simulink model "Project_UR5"  (Simulink 8.3)
settings: Solver=ode3  StartTime=0.0  StopTime=tf  FixedStep=ts  RelTol=1e-3
values from neighbouring files (symbols this model uses):
  qi = [0;pi/4;0;-pi/3;0;0]    [initial.m]
(part 2 of 3)

== matlab function Inverse Kinematics & Redundant Kinematic Controller ==
  data: x_des input double; dq output double; xd_des input double; q input double
function dq = IK_Control(x_des,xd_des,q)
%Input Decomposition
q1 = q(1);
q2 = q(2);
q3 = q(3);
q4 = q(4);
q5 = q(5);
q6 = q(6);
%% %% Inverse Kinematics
%% End Effector Position
x = [(379*cos(q2 + q3)*cos(q1)*sin(q4))/4 - 425*cos(q1)*cos(q2) - (165*cos(q5)*sin(q1))/2 - (165*cos(q2 + q3 + q4)*cos(q1)*sin(q5))/2 - (1093*sin(q1))/10 + (379*sin(q2 + q3)*cos(q1)*cos(q4))/4 - 392*cos(q1)*cos(q2)*cos(q3) + 392*cos(q1)*sin(q2)*sin(q3);
(1093*cos(q1))/10 + (165*cos(q1)*cos(q5))/2 - 425*cos(q2)*sin(q1) + 392*sin(q1)*sin(q2)*sin(q3) - (165*cos(q2 + q3 + q4)*sin(q1)*sin(q5))/2 + (379*cos(q2 + q3)*sin(q1)*sin(q4))/4 + (379*sin(q2 + q3)*cos(q4)*sin(q1))/4 - 392*cos(q2)*cos(q3)*sin(q1);
392*sin(q2 + q3) + 425*sin(q2) + sin(q5)*((165*cos(q2 + q3)*sin(q4))/2 + (165*sin(q2 + q3)*cos(q4))/2) + (379*cos(q2 + q3)*cos(q4))/4 - (379*sin(q2 + q3)*sin(q4))/4 + 446/5];

%% Jacobian 6x6
J = [ 425*cos(q2)*sin(q1) - (165*cos(q1)*cos(q5))/2 - (1093*cos(q1))/10 - 392*sin(q1)*sin(q2)*sin(q3) + (165*cos(q2 + q3 + q4)*sin(q1)*sin(q5))/2 - (379*cos(q2 + q3)*sin(q1)*sin(q4))/4 - (379*sin(q2 + q3)*cos(q4)*sin(q1))/4 + 392*cos(q2)*cos(q3)*sin(q1), cos(q1)*(392*sin(q2 + q3) + 425*sin(q2) + sin(q5)*((165*cos(q2 + q3)*sin(q4))/2 + (165*sin(q2 + q3)*cos(q4))/2) + (379*cos(q2 + q3)*cos(q4))/4 - (379*sin(q2 + q3)*sin(q4))/4),                     cos(q1)*((379*cos(q2 + q3 + q4))/4 + 392*sin(q2 + q3) + (165*sin(q2 + q3 + q4)*sin(q5))/2),                     cos(q1)*((379*cos(q2 + q3 + q4))/4 + (165*sin(q2 + q3 + q4)*sin(q5))/2), (165*sin(q1)*sin(q5))/2 - (165*cos(q1)*cos(q2)*cos(q3)*cos(q4)*cos(q5))/2 + (165*cos(q1)*cos(q2)*cos(q5)*sin(q3)*sin(q4))/2 + (165*cos(q1)*cos(q3)*cos(q5)*sin(q2)*sin(q4))/2 + (165*cos(q1)*cos(q4)*cos(q5)*sin(q2)*sin(q3))/2,                                                     0;
 (379*cos(q2 + q3)*cos(q1)*sin(q4))/4 - 425*cos(q1)*cos(q2) - (165*cos(q5)*sin(q1))/2 - (165*cos(q2 + q3 + q4)*cos(q1)*sin(q5))/2 - (1093*sin(q1))/10 + (379*sin(q2 + q3)*cos(q1)*cos(q4))/4 - 392*cos(q1)*cos(q2)*cos(q3) + 392*cos(q1)*sin(q2)*sin(q3), sin(q1)*(392*sin(q2 + q3) + 425*sin(q2) + sin(q5)*((165*cos(q2 + q3)*sin(q4))/2 + (165*sin(q2 + q3)*cos(q4))/2) + (379*cos(q2 + q3)*cos(q4))/4 - (379*sin(q2 + q3)*sin(q4))/4),                     sin(q1)*((379*cos(q2 + q3 + q4))/4 + 392*sin(q2 + q3) + (165*sin(q2 + q3 + q4)*sin(q5))/2),                     sin(q1)*((379*cos(q2 + q3 + q4))/4 + (165*sin(q2 + q3 + q4)*sin(q5))/2), (165*cos(q2)*cos(q5)*sin(q1)*sin(q3)*sin(q4))/2 - (165*cos(q2)*cos(q3)*cos(q4)*cos(q5)*sin(q1))/2 - (165*cos(q1)*sin(q5))/2 + (165*cos(q3)*cos(q5)*sin(q1)*sin(q2)*sin(q4))/2 + (165*cos(q4)*cos(q5)*sin(q1)*sin(q2)*sin(q3))/2,                                                     0;
                                                                                                                                                                                                                                                       0,                                                   (165*sin(q2 + q3 + q4 + q5))/4 - (379*sin(q2 + q3 + q4))/4 + 392*cos(q2 + q3) + 425*cos(q2) - (165*sin(q2 + q3 + q4 - q5))/4, (165*sin(q2 + q3 + q4 + q5))/4 - (379*sin(q2 + q3 + q4))/4 + 392*cos(q2 + q3) - (165*sin(q2 + q3 + q4 - q5))/4, (165*sin(q2 + q3 + q4 + q5))/4 - (379*sin(q2 + q3 + q4))/4 - (165*sin(q2 + q3 + q4 - q5))/4,                                                                                                                                                                 (165*sin(q2 + q3 + q4 + q5))/4 + (165*sin(q2 + q3 + q4 - q5))/4,                                                     0;
                                                                                                                                                                                                                                                       0,                                                                                                                                                                       -sin(q1),                                                                                                       -sin(q1),                                                                                    -sin(q1),                                                                                                                                                                                                       sin(q2 + q3 + q4)*cos(q1), - cos(q5)*sin(q1) - cos(q2 + q3 + q4)*cos(q1)*sin(q5);
                                                                                                                                                                                                                                                       0,                                                                                                                                                                        cos(q1),                                                                                                        cos(q1),                                                                                     cos(q1),                                                                                                                                                                                                       sin(q2 + q3 + q4)*sin(q1),   cos(q1)*cos(q5) - cos(q2 + q3 + q4)*sin(q1)*sin(q5);
                                                                                                                                                                                                                                                       1,                                                                                                                                                                              0,                                                                                                              0,                                                                                           0,                                                                                                                                                                                                               cos(q2 + q3 + q4),                             sin(q2 + q3 + q4)*sin(q5)];

%% Redundant Jacobian 3x6
Jp=J(1:3,1:6) ; %% Task only takes 3 DOFs to control x,y,z.

% %% manipulability measure #1: W=det(Jp*Jp.')
% kp=0.001;
% dq0=[0;
%    -(2^(1/2)*(317026377437840000*cos(2*q2 + q4) - 1082343818118750000*cos(2*q2 - q3 - q4 - q5) - 41912575773750000*cos(2*q2 - q3 - q4 - 2*q5) + 16565733236250000*cos(2*q2 - q3 - q4 + 2*q5) - 540213828000000000*cos(2*q2 - 2*q3 - q4 - q5) + 396576415666421760*cos(2*q2 + 2*q3 - q4 - q5) + 16552357593750000*cos(2*q2 - q3 - q4 - 3*q5) - 16552357593750000*cos(2*q2 - q3 - q4 + 3*q5) - 45886635629936640*cos(2*q2 + 2*q3 - q4 - 2*q5) + 45886635629936640*cos(2*q2 + 2*q3 - q4 + 2*q5) + 17317691854848000*cos(2*q2 + 2*q3 - q4 - 3*q5) - 17317691854848000*cos(2*q2 + 2*q3 - q4 + 3*q5) + 192863414377307520*cos(2*q2 + 2*q3 + 3*q4 - q5) + 139667883829911360*cos(2*q2 + 2*q3 + 3*q4 - 2*q5) + 136338643638267840*cos(2*q2 + 2*q3 + 3*q4 + 2*q5) + 275626326313503000*cos(2*q2 + 3*q3 + 3*q4 - q5) + 34919056932883200*cos(2*q2 + 2*q3 + 3*q4 - 3*q5) - 30250558196812800*cos(2*q2 + 2*q3 + 3*q4 + 3*q5) + 175870104928699500*cos(2*q2 + 3*q3 + 3*q4 - 2*q5) + 174065350998280500*cos(2*q2 + 3*q3 + 3*q4 + 2*q5) + 200938795318800000*cos(2*q2 + 4*q3 + 3*q4 - q5) + 508114967976000*cos(2*q2 + 2*q3 + 3*q4 - 4*q5) - 508114967976000*cos(2*q2 + 2*q3 + 3*q4 + 4*q5) + 36593293892265000*cos(2*q2 + 3*q3 + 3*q4 - 3*q5) - 34062538837635000*cos(2*q2 + 3*q3 + 3*q4 + 3*q5) + 116893673820000000*cos(2*q2 + 4*q3 + 3*q4 - 2*q5) + 116893673820000000*cos(2*q2 + 4*q3 + 3*q4 + 2*q5) + 275444976262500*cos(2*q2 + 3*q3 + 3*q4 - 4*q5) - 275444976262500*cos(2*q2 + 3*q3 + 3*q4 + 4*q5) + 20356154280000000*cos(2*q2 + 4*q3 + 3*q4 - 3*q5) - 20356154280000000*cos(2*q2 + 4*q3 + 3*q4 + 3*q5) + 14526380593972122400*sin(2*q2 + q3) - 4445768516062500*sin(2*q2 + q5) - 722615438160000000*sin(2*q2 - q3 - 2*q4 - q5) + 262162593000000000*sin(2*q2 - q3 - 2*q4 - 2*q5) + 262162593000000000*sin(2*q2 - q3 - 2*q4 + 2*q5) - 261149286750000000*sin(2*q2 - 2*q3 - 2*q4 - q5) - 189006783727534080*sin(2*q2 + 2*q3 - 2*q4 - q5) + 127716498108106380*sin(2*q2 + 2*q3 + 2*q4 - q5) + 85269720937500000*sin(2*q2 - 2*q3 - 2*q4 - 2*q5) + 85269720937500000*sin(2*q2 - 2*q3 - 2*q4 + 2*q5) + 82285275237580800*sin(2*q2 + 2*q3 - 2*q4 - 2*q5) + 82285275237580800*sin(2*q2 + 2*q3 - 2*q4 + 2*q5) + 235845517878338346*sin(2*q2 + 2*q3 + 2*q4 - 2*q5) + 165406186902402666*sin(2*q2 + 2*q3 + 2*q4 + 2*q5) + 1142121750227304000*sin(2*q2 + 3*q3 + 2*q4 - q5) + 18769510446883020*sin(2*q2 + 2*q3 + 2*q4 - 3*q5) + 11896689054513780*sin(2*q2 + 2*q3 + 2*q4 + 3*q5) - 11620198292989440*sin(2*q2 + 2*q3 + 4*q4 - q5) + 358818080264028000*sin(2*q2 + 3*q3 + 2*q4 - 2*q5) + 334768238290332000*sin(2*q2 + 3*q3 + 2*q4 + 2*q5) + 777590887180800000*sin(2*q2 + 4*q3 + 2*q4 - q5) + 748031352071850*sin(2*q2 + 2*q3 + 2*q4 - 4*q5) + 748031352071850*sin(2*q2 + 2*q3 + 2*q4 + 4*q5) - 15003495465235200*sin(2*q2 + 2*q3 + 4*q4 - 2*q5) - 15003495465235200*sin(2*q2 + 2*q3 + 4*q4 + 2*q5) + 5235123912480000*sin(2*q2 + 3*q3 + 2*q4 - 3*q5) + 5235123912480000*sin(2*q2 + 3*q3 + 2*q4 + 3*q5) - 12598429271736000*sin(2*q2 + 3*q3 + 4*q4 - q5) + 193445150976000000*sin(2*q2 + 4*q3 + 2*q4 - 2*q5) + 193445150976000000*sin(2*q2 + 4*q3 + 2*q4 + 2*q5) - 6278767742016000*sin(2*q2 + 2*q3 + 4*q4 - 3*q5) + 6278767742016000*sin(2*q2 + 2*q3 + 4*q4 + 3*q5) - 16266544828380000*sin(2*q2 + 3*q3 + 4*q4 - 2*q5) - 16266544828380000*sin(2*q2 + 3*q3 + 4*q4 + 2*q5) - 12428943969337500*sin(2*q2 + 4*q3 + 4*q4 - q5) - 911166822720000*sin(2*q2 + 2*q3 + 4*q4 - 4*q5) - 911166822720000*sin(2*q2 + 2*q3 + 4*q4 + 4*q5) - 6807337475400000*sin(2*q2 + 3*q3 + 4*q4 - 3*q5) + 6807337475400000*sin(2*q2 + 3*q3 + 4*q4 + 3*q5) - 16223208602906250*sin(2*q2 + 4*q3 + 4*q4 - 2*q5) - 16223208602906250*sin(2*q2 + 4*q3 + 4*q4 + 2*q5) - 987872193000000*sin(2*q2 + 3*q3 + 4*q4 - 4*q5) - 987872193000000*sin(2*q2 + 3*q3 + 4*q4 + 4*q5) - 6150336792187500*sin(2*q2 + 4*q3 + 4*q4 - 3*q5) + 6150336792187500*sin(2*q2 + 4*q3 + 4*q4 + 3*q5) - 803276177343750*sin(2*q2 + 4*q3 + 4*q4 - 4*q5) - 803276177343750*sin(2*q2 + 4*q3 + 4*q4 + 4*q5) + 2498784373190000000*cos(2*q2 - q3 - q4) + 1240854792800000000*cos(2*q2 - 2*q3 - q4) - 871145795906584576*cos(2*q2 + 2*q3 - q4) - 62388715527600000*cos(2*q2 - q4 - q5) + 63675071524036224*cos(2*q2 + 2*q3 + 3*q4) - 92595827847600000*cos(2*q2 - q4 - 2*q5) + 69217093083600000*cos(2*q2 - q4 + 2*q5) + 45801347130000000*cos(2*q2 - q4 - 3*q5) - 45801347130000000*cos(2*q2 - q4 + 3*q5) + 34513957880105600*cos(2*q2 + 3*q3 + 3*q4) - 2008123829040000*cos(2*q2 + 4*q3 + 3*q4) + 4969165728210312500*sin(2*q2) + 725047844808000000*sin(2*q2 - q3 - 2*q4) + 104865037200000000*sin(2*q2 - q3 - 2*q5) + 104865037200000000*sin(2*q2 - q3 + 2*q5) + 243079518400000000*sin(2*q2 - 2*q3 - 2*q4) + 217071427371925504*sin(2*q2 + 2*q3 - 2*q4) + 438536338768182720*sin(2*q2 + 2*q3 + 2*q4) - 11750186456870400*sin(2*q2 + 2*q3 - q5) - 131469808648502016*sin(2*q2 + 2*q3 - 2*q5) - 175834693607037696*sin(2*q2 + 2*q3 + 2*q5) + 1012290445559159200*sin(2*q2 + 3*q3 + 2*q4) - 888675299635200000*sin(2*q2 - 2*q4 - q5) + 333253237363200000*sin(2*q2 + 2*q4 - q5) + 9532529563768064*sin(2*q2 + 2*q3 + 4*q4) + 7564341295526400*sin(2*q2 + 2*q3 - 3*q5) + 11750186456870400*sin(2*q2 + 2*q3 + 3*q5) + 362709658080000000*sin(2*q2 - 2*q4 - 2*q5) + 362709658080000000*sin(2*q2 - 2*q4 + 2*q5) + 120903219360000000*sin(2*q2 + 2*q4 - 2*q5) + 120903219360000000*sin(2*q2 + 2*q4 + 2*q5) + 602883625783040000*sin(2*q2 + 4*q3 + 2*q4) - 1822333645440000*sin(2*q2 + 2*q3 - 4*q5) - 1822333645440000*sin(2*q2 + 2*q3 + 4*q5) + 10335012919901600*sin(2*q2 + 3*q3 + 4*q4) + 13494962268852500*sin(2*q2 + 4*q3 + 4*q4) + 2457973257707649000*cos(2*q2 + q3 + q4 - q5) - 869311129682688000*cos(2*q2 + q3 - q4 + q5) + 498267813120000000*cos(2*q2 - q3 + q4 + q5) - 133864358657663700*cos(2*q2 + q3 + q4 - 2*q5) + 76464939583365300*cos(2*q2 + q3 + q4 + 2*q5) - 1325918940020727360*cos(2*q2 + 2*q3 + q4 + q5) + 689315467203000*cos(2*q2 + q3 + q4 - 3*q5) + 6902949696687000*cos(2*q2 + q3 + q4 + 3*q5) - 129816178829568000*cos(2*q2 + q3 + 3*q4 + q5) + 1407721742617344000*cos(2*q2 + 3*q3 + q4 + q5) + 1377224881312500*cos(2*q2 + q3 + q4 - 4*q5) - 1377224881312500*cos(2*q2 + q3 + q4 + 4*q5) + 919157565849600000*cos(2*q2 + 4*q3 + q4 + q5) + 614754207277056000*sin(2*q2 + q3 - 2*q4 + q5) - 153499453009056000*sin(2*q2 + q3 + 2*q4 + q5) + 225130560673760000*cos(2*q2 - q4) - 5011691754440000000*sin(2*q2 - q3) - 2566834188800000000*sin(2*q2 - 2*q3) + 4963773870401251584*sin(2*q2 + 2*q3) - 4321284125611622400*sin(2*q2 + 3*q3) + 972268829109760000*sin(2*q2 - 2*q4) + 334375006076160000*sin(2*q2 + 2*q4) - 6905903232937500*sin(2*q2 - q5) - 2183695550382080000*sin(2*q2 + 4*q3) + 51773906290713750*sin(2*q2 - 2*q5) + 25699460273313750*sin(2*q2 + 2*q5) + 4445768516062500*sin(2*q2 - 3*q5) + 6905903232937500*sin(2*q2 + 3*q5) - 2945345983593750*sin(2*q2 - 4*q5) - 2945345983593750*sin(2*q2 + 4*q5) + 5604346536115055200*cos(2*q2 + q3 + q4) - 143108437718400000*cos(2*q2 + q4 + q5) - 13784708710080000*sin(2*q2 + q3 + q5) + 869311129682688000*cos(2*q2 + q3 - q4 - q5) - 498267813120000000*cos(2*q2 - q3 + q4 - q5) + 1082343818118750000*cos(2*q2 - q3 - q4 + q5) - 99499082360832000*cos(2*q2 + q3 - q4 - 2*q5) + 99499082360832000*cos(2*q2 + q3 - q4 + 2*q5) + 540213828000000000*cos(2*q2 - 2*q3 - q4 + q5) + 1318916191916621760*cos(2*q2 + 2*q3 + q4 - q5) - 396576415666421760*cos(2*q2 + 2*q3 - q4 + q5) + 46938896928000000*cos(2*q2 + q3 - q4 - 3*q5) - 46938896928000000*cos(2*q2 + q3 - q4 + 3*q5) + 129816178829568000*cos(2*q2 + q3 + 3*q4 - q5) - 140429041403466816*cos(2*q2 + 2*q3 + q4 - 2*q5) + 57922730157466944*cos(2*q2 + 2*q3 + q4 + 2*q5) - 1407721742617344000*cos(2*q2 + 3*q3 + q4 - q5) + 86253779082240000*cos(2*q2 + q3 + 3*q4 - 2*q5) + 86253779082240000*cos(2*q2 + q3 + 3*q4 + 2*q5) - 14458443039754560*cos(2*q2 + 2*q3 + q4 - 3*q5) + 21461191143860160*cos(2*q2 + 2*q3 + q4 + 3*q5) - 197531913113377920*cos(2*q2 + 2*q3 + 3*q4 + q5) - 24874770590208000*cos(2*q2 + 3*q3 + q4 - 2*q5) + 24874770590208000*cos(2*q2 + 3*q3 + q4 + 2*q5) - 919157565849600000*cos(2*q2 + 4*q3 + q4 - q5) + 18775558771200000*cos(2*q2 + q3 + 3*q4 - 3*q5) - 18775558771200000*cos(2*q2 + q3 + 3*q4 + 3*q5) + 1016229935952000*cos(2*q2 + 2*q3 + q4 - 4*q5) - 1016229935952000*cos(2*q2 + 2*q3 + q4 + 4*q5) - 278157081368133000*cos(2*q2 + 3*q3 + 3*q4 + q5) - 200938795318800000*cos(2*q2 + 4*q3 + 3*q4 + q5) - 614754207277056000*sin(2*q2 + q3 - 2*q4 - q5) + 137794081271616000*sin(2*q2 + q3 + 2*q4 - q5) + 722615438160000000*sin(2*q2 - q3 - 2*q4 + q5) + 267637055938560000*sin(2*q2 + q3 - 2*q4 - 2*q5) + 267637055938560000*sin(2*q2 + q3 - 2*q4 + 2*q5) + 191880299736972000*sin(2*q2 + q3 + 2*q4 - 2*q5) + 155805536776428000*sin(2*q2 + q3 + 2*q4 + 2*q5) + 261149286750000000*sin(2*q2 - 2*q3 - 2*q4 + q5) + 189006783727534080*sin(2*q2 + 2*q3 - 2*q4 + q5) - 158382697609503180*sin(2*q2 + 2*q3 + 2*q4 + q5) + 5583573376920000*sin(2*q2 + q3 + 2*q4 - 3*q5) + 10121798360520000*sin(2*q2 + q3 + 2*q4 + 3*q5) - 1152591998052264000*sin(2*q2 + 3*q3 + 2*q4 + q5) - 987872193000000*sin(2*q2 + q3 + 2*q4 - 4*q5) - 987872193000000*sin(2*q2 + q3 + 2*q4 + 4*q5) + 11620198292989440*sin(2*q2 + 2*q3 + 4*q4 + q5) - 777590887180800000*sin(2*q2 + 4*q3 + 2*q4 + q5) + 12598429271736000*sin(2*q2 + 3*q3 + 4*q4 + q5) + 12428943969337500*sin(2*q2 + 4*q3 + 4*q4 + q5) - 1888964098266828800*cos(2*q2 + q3 - q4) - 1144506067712000000*cos(2*q2 - q3 + q4) + 2996299920147470720*cos(2*q2 + 2*q3 + q4) + 27516460414105600*cos(2*q2 + q3 + 3*q4) + 143108437718400000*cos(2*q2 + q4 - q5) + 62388715527600000*cos(2*q2 - q4 + q5) - 3233494184557414400*cos(2*q2 + 3*q3 + q4) - 15279452773200000*cos(2*q2 + q4 - 2*q5) + 38658187537200000*cos(2*q2 + q4 + 2*q5) - 2111277075496960000*cos(2*q2 + 4*q3 + q4) + 15267115710000000*cos(2*q2 + q4 - 3*q5) - 15267115710000000*cos(2*q2 + q4 + 3*q5) + 706035892600012800*sin(2*q2 + q3 - 2*q4) + 390748536798496800*sin(2*q2 + q3 + 2*q4) - 22861158677280000*sin(2*q2 + q3 - q5) - 188957478197426400*sin(2*q2 + q3 - 2*q5) - 249082083131666400*sin(2*q2 + q3 + 2*q5) - 7564341295526400*sin(2*q2 + 2*q3 + q5) + 13784708710080000*sin(2*q2 + q3 - 3*q5) + 22861158677280000*sin(2*q2 + q3 + 3*q5) + 888675299635200000*sin(2*q2 - 2*q4 + q5) - 333253237363200000*sin(2*q2 + 2*q4 + q5) - 3951488772000000*sin(2*q2 + q3 - 4*q5) - 3951488772000000*sin(2*q2 + q3 + 4*q5) - 2465565522871539000*cos(2*q2 + q3 + q4 + q5)))/(128*(7263190296986061200*cos(2*q2 + q3) + 235345297533337600*cos(q3 - 2*q4) + 822231539407213600*cos(q3 + 2*q4) - 10296023092740000*cos(q3 - q5) - 2222884258031250*cos(2*q2 + q5) - 70107391443751200*cos(q3 - 2*q5) - 76119851937175200*cos(q3 + 2*q5) + 8026910600940000*cos(q3 - 3*q5) + 10296023092740000*cos(q3 + 3*q5) - 445882949398656000*cos(2*q4 + q5) - 493936096500000*cos(q3 - 4*q5) - 493936096500000*cos(q3 + 4*q5) - 361307719080000000*cos(2*q2 - q3 - 2*q4 - q5) + 131081296500000000*cos(2*q2 - q3 - 2*q4 - 2*q5) + 131081296500000000*cos(2*q2 - q3 - 2*q4 + 2*q5) - 130574643375000000*cos(2*q2 - 2*q3 - 2*q4 - q5) - 94503391863767040*cos(2*q2 + 2*q3 - 2*q4 - q5) + 63858249054053190*cos(2*q2 + 2*q3 + 2*q4 - q5) + 42634860468750000*cos(2*q2 - 2*q3 - 2*q4 - 2*q5) + 42634860468750000*cos(2*q2 - 2*q3 - 2*q4 + 2*q5) + 41142637618790400*cos(2*q2 + 2*q3 - 2*q4 - 2*q5) + 41142637618790400*cos(2*q2 + 2*q3 - 2*q4 + 2*q5) + 117922758939169173*cos(2*q2 + 2*q3 + 2*q4 - 2*q5) + 82703093451201333*cos(2*q2 + 2*q3 + 2*q4 + 2*q5) + 571060875113652000*cos(2*q2 + 3*q3 + 2*q4 - q5) + 9384755223441510*cos(2*q2 + 2*q3 + 2*q4 - 3*q5) + 5948344527256890*cos(2*q2 + 2*q3 + 2*q4 + 3*q5) - 5810099146494720*cos(2*q2 + 2*q3 + 4*q4 - q5) + 179409040132014000*cos(2*q2 + 3*q3 + 2*q4 - 2*q5) + 167384119145166000*cos(2*q2 + 3*q3 + 2*q4 + 2*q5) + 388795443590400000*cos(2*q2 + 4*q3 + 2*q4 - q5) + 374015676035925*cos(2*q2 + 2*q3 + 2*q4 - 4*q5) + 374015676035925*cos(2*q2 + 2*q3 + 2*q4 + 4*q5) - 7501747732617600*cos(2*q2 + 2*q3 + 4*q4 - 2*q5) - 7501747732617600*cos(2*q2 + 2*q3 + 4*q4 + 2*q5) + 2617561956240000*cos(2*q2 + 3*q3 + 2*q4 - 3*q5) + 2617561956240000*cos(2*q2 + 3*q3 + 2*q4 + 3*q5) - 6299214635868000*cos(2*q2 + 3*q3 + 4*q4 - q5) + 96722575488000000*cos(2*q2 + 4*q3 + 2*q4 - 2*q5) + 96722575488000000*cos(2*q2 + 4*q3 + 2*q4 + 2*q5) - 3139383871008000*cos(2*q2 + 2*q3 + 4*q4 - 3*q5) + 3139383871008000*cos(2*q2 + 2*q3 + 4*q4 + 3*q5) - 8133272414190000*cos(2*q2 + 3*q3 + 4*q4 - 2*q5) - 8133272414190000*cos(2*q2 + 3*q3 + 4*q4 + 2*q5) - 6214471984668750*cos(2*q2 + 4*q3 + 4*q4 - q5) - 455583411360000*cos(2*q2 + 2*q3 + 4*q4 - 4*q5) - 455583411360000*cos(2*q2 + 2*q3 + 4*q4 + 4*q5) - 3403668737700000*cos(2*q2 + 3*q3 + 4*q4 - 3*q5) + 3403668737700000*cos(2*q2 + 3*q3 + 4*q4 + 3*q5) - 8111604301453125*cos(2*q2 + 4*q3 + 4*q4 - 2*q5) - 8111604301453125*cos(2*q2 + 4*q3 + 4*q4 + 2*q5) - 493936096500000*cos(2*q2 + 3*q3 + 4*q4 - 4*q5) - 493936096500000*cos(2*q2 + 3*q3 + 4*q4 + 4*q5) - 3075168396093750*cos(2*q2 + 4*q3 + 4*q4 - 3*q5) + 3075168396093750*cos(2*q2 + 4*q3 + 4*q4 + 3*q5) - 401638088671875*cos(2*q2 + 4*q3 + 4*q4 - 4*q5) - 401638088671875*cos(2*q2 + 4*q3 + 4*q4 + 4*q5) + 572253033856000000*sin(q3 - q4) - 158513188718920000*sin(2*q2 + q4) + 2944433354427040000*sin(2*q3 + q4) - 27516460414105600*sin(q3 + 3*q4) - 1693976898423939360*sin(q4 - q5) + 1716759101568000000*sin(3*q3 + q4) + 153879467142538368*sin(q4 - 2*q5) - 54179474609538432*sin(q4 + 2*q5) - 7896057578529120*sin(q4 - 3*q5) + 6728932894511520*sin(q4 + 3*q5) + 59868167177871360*sin(q5 - 3*q4) + 59868167177871360*sin(3*q4 + q5) - 762172451964000*sin(q4 - 4*q5) + 762172451964000*sin(q4 + 4*q5) + 541171909059375000*sin(2*q2 - q3 - q4 - q5) + 20956287886875000*sin(2*q2 - q3 - q4 - 2*q5) - 8282866618125000*sin(2*q2 - q3 - q4 + 2*q5) + 270106914000000000*sin(2*q2 - 2*q3 - q4 - q5) - 198288207833210880*sin(2*q2 + 2*q3 - q4 - q5) - 8276178796875000*sin(2*q2 - q3 - q4 - 3*q5) + 8276178796875000*sin(2*q2 - q3 - q4 + 3*q5) + 22943317814968320*sin(2*q2 + 2*q3 - q4 - 2*q5) - 22943317814968320*sin(2*q2 + 2*q3 - q4 + 2*q5) - 8658845927424000*sin(2*q2 + 2*q3 - q4 - 3*q5) + 8658845927424000*sin(2*q2 + 2*q3 - q4 + 3*q5) - 96431707188653760*sin(2*q2 + 2*q3 + 3*q4 - q5) - 69833941914955680*sin(2*q2 + 2*q3 + 3*q4 - 2*q5) - 68169321819133920*sin(2*q2 + 2*q3 + 3*q4 + 2*q5) - 137813163156751500*sin(2*q2 + 3*q3 + 3*q4 - q5) - 17459528466441600*sin(2*q2 + 2*q3 + 3*q4 - 3*q5) + 15125279098406400*sin(2*q2 + 2*q3 + 3*q4 + 3*q5) - 87935052464349750*sin(2*q2 + 3*q3 + 3*q4 - 2*q5) - 87032675499140250*sin(2*q2 + 3*q3 + 3*q4 + 2*q5) - 100469397659400000*sin(2*q2 + 4*q3 + 3*q4 - q5) - 254057483988000*sin(2*q2 + 2*q3 + 3*q4 - 4*q5) + 254057483988000*sin(2*q2 + 2*q3 + 3*q4 + 4*q5) - 18296646946132500*sin(2*q2 + 3*q3 + 3*q4 - 3*q5) + 17031269418817500*sin(2*q2 + 3*q3 + 3*q4 + 3*q5) - 58446836910000000*sin(2*q2 + 4*q3 + 3*q4 - 2*q5) - 58446836910000000*sin(2*q2 + 4*q3 + 3*q4 + 2*q5) - 137722488131250*sin(2*q2 + 3*q3 + 3*q4 - 4*q5) + 137722488131250*sin(2*q2 + 3*q3 + 3*q4 + 4*q5) - 10178077140000000*sin(2*q2 + 4*q3 + 3*q4 - 3*q5) + 10178077140000000*sin(2*q2 + 4*q3 + 3*q4 + 3*q5) + 656825094627009000*sin(q3 + q4 + q5) + 2484582864105156250*cos(2*q2) - 4926469791532800000*cos(2*q3) - 2367527063552000000*cos(3*q3) + 588766372249655040*cos(2*q4) - 427286086914756762*cos(2*q5) + 15333099750698400*cos(3*q5) + 1659198174791850*cos(4*q5) + 362523922404000000*cos(2*q2 - q3 - 2*q4) + 52432518600000000*cos(2*q2 - q3 - 2*q5) + 52432518600000000*cos(2*q2 - q3 + 2*q5) + 121539759200000000*cos(2*q2 - 2*q3 - 2*q4) + 108535713685962752*cos(2*q2 + 2*q3 - 2*q4) + 219268169384091360*cos(2*q2 + 2*q3 + 2*q4) - 5875093228435200*cos(2*q2 + 2*q3 - q5) - 65734904324251008*cos(2*q2 + 2*q3 - 2*q5) - 87917346803518848*cos(2*q2 + 2*q3 + 2*q5) + 506145222779579600*cos(2*q2 + 3*q3 + 2*q4) - 444337649817600000*cos(2*q2 - 2*q4 - q5) + 166626618681600000*cos(2*q2 + 2*q4 - q5) + 4766264781884032*cos(2*q2 + 2*q3 + 4*q4) + 3782170647763200*cos(2*q2 + 2*q3 - 3*q5) + 5875093228435200*cos(2*q2 + 2*q3 + 3*q5) + 181354829040000000*cos(2*q2 - 2*q4 - 2*q5) + 181354829040000000*cos(2*q2 - 2*q4 + 2*q5) + 60451609680000000*cos(2*q2 + 2*q4 - 2*q5) + 60451609680000000*cos(2*q2 + 2*q4 + 2*q5) + 301441812891520000*cos(2*q2 + 4*q3 + 2*q4) + 959938898447100000*cos(2*q3 + 2*q4 - q5) - 911166822720000*cos(2*q2 + 2*q3 - 4*q5) - 911166822720000*cos(2*q2 + 2*q3 + 4*q5) + 5167506459950800*cos(2*q2 + 3*q3 + 4*q4) + 311602195537256250*cos(2*q3 + 2*q4 - 2*q5) + 298564972528556250*cos(2*q3 + 2*q4 + 2*q5) + 481743625440000000*cos(3*q3 + 2*q4 - q5) + 6747481134426250*cos(2*q2 + 4*q3 + 4*q4) - 4542486213375000*cos(2*q3 + 2*q4 - 3*q5) + 10218322087875000*cos(2*q3 + 2*q4 + 3*q5) + 131081296500000000*cos(3*q3 + 2*q4 - 2*q5) + 131081296500000000*cos(3*q3 + 2*q4 + 2*q5) - 1874311080468750*cos(2*q3 + 2*q4 - 4*q5) - 1874311080468750*cos(2*q3 + 2*q4 + 4*q5) - 12689944096858112*sin(3*q4) - 1249392186595000000*sin(2*q2 - q3 - q4) - 620427396400000000*sin(2*q2 - 2*q3 - q4) + 435572897953292288*sin(2*q2 + 2*q3 - q4) + 31194357763800000*sin(2*q2 - q4 - q5) - 31837535762018112*sin(2*q2 + 2*q3 + 3*q4) + 46297913923800000*sin(2*q2 - q4 - 2*q5) - 34608546541800000*sin(2*q2 - q4 + 2*q5) + 229789391462400000*sin(2*q3 - q4 - q5) - 22900673565000000*sin(2*q2 - q4 - 3*q5) + 22900673565000000*sin(2*q2 - q4 + 3*q5) - 17256978940052800*sin(2*q2 + 3*q3 + 3*q4) + 1004061914520000*sin(2*q2 + 4*q3 + 3*q4) - 138200062354200000*sin(2*q3 + 3*q4 - q5) - 87670255365000000*sin(2*q3 + 3*q4 - 2*q5) - 87670255365000000*sin(2*q3 + 3*q4 + 2*q5) - 73537762505625000*sin(3*q3 + 3*q4 - q5) - 17811634995000000*sin(2*q3 + 3*q4 - 3*q5) + 17811634995000000*sin(2*q3 + 3*q4 + 3*q5) - 44356974440625000*sin(3*q3 + 3*q4 - 2*q5) - 44356974440625000*sin(3*q3 + 3*q4 + 2*q5) - 8276178796875000*sin(3*q3 + 3*q4 - 3*q5) + 8276178796875000*sin(3*q3 + 3*q4 + 3*q5) + 307377103638528000*cos(2*q2 + q3 - 2*q4 + q5) - 76749726504528000*cos(2*q2 + q3 + 2*q4 + q5) - 1228986628853824500*sin(2*q2 + q3 + q4 - q5) + 434655564841344000*sin(2*q2 + q3 - q4 + q5) - 249133906560000000*sin(2*q2 - q3 + q4 + q5) + 66932179328831850*sin(2*q2 + q3 + q4 - 2*q5) - 38232469791682650*sin(2*q2 + q3 + q4 + 2*q5) + 662959470010363680*sin(2*q2 + 2*q3 + q4 + q5) - 344657733601500*sin(2*q2 + q3 + q4 - 3*q5) - 3451474848343500*sin(2*q2 + q3 + q4 + 3*q5) + 64908089414784000*sin(2*q2 + q3 + 3*q4 + q5) - 703860871308672000*sin(2*q2 + 3*q3 + q4 + q5) - 688612440656250*sin(2*q2 + q3 + q4 - 4*q5) + 688612440656250*sin(2*q2 + q3 + q4 + 4*q5) - 459578782924800000*sin(2*q2 + 4*q3 + q4 + q5) - 2505845877220000000*cos(2*q2 - q3) - 1283417094400000000*cos(2*q2 - 2*q3) + 2481886935200625792*cos(2*q2 + 2*q3) - 2160642062805811200*cos(2*q2 + 3*q3) + 486134414554880000*cos(2*q2 - 2*q4) + 167187503038080000*cos(2*q2 + 2*q4) - 3452951616468750*cos(2*q2 - q5) - 1091847775191040000*cos(2*q2 + 4*q3) + 25886953145356875*cos(2*q2 - 2*q5) + 12849730136656875*cos(2*q2 + 2*q5) + 883398735766092500*cos(2*q3 + 2*q4) + 2222884258031250*cos(2*q2 - 3*q5) + 3452951616468750*cos(2*q2 + 3*q5) + 120903219360000000*cos(2*q3 - 2*q5) + 120903219360000000*cos(2*q3 + 2*q5) + 395977698872000000*cos(3*q3 + 2*q4) + 436225685522457600*cos(2*q4 - q5) - 1472672991796875*cos(2*q2 - 4*q5) - 1472672991796875*cos(2*q2 + 4*q5) + 241523670772581120*cos(2*q4 - 2*q5) + 219341228293313280*cos(2*q4 + 2*q5) - 1450135803916800*cos(2*q4 - 3*q5) + 11107399680115200*cos(2*q4 + 3*q5) - 1822333645440000*cos(2*q4 - 4*q5) - 1822333645440000*cos(2*q4 + 4*q5) - 112565280336880000*sin(2*q2 - q4) - 527819268874240000*sin(2*q3 - q4) - 18143529750640000*sin(2*q3 + 3*q4) - 3498748733000000*sin(3*q3 + 3*q4) - 39778213412044800*sin(3*q4 - 2*q5) - 39778213412044800*sin(3*q4 + 2*q5) - 8658845927424000*sin(3*q4 - 3*q5) + 8658845927424000*sin(3*q4 + 3*q5) - 6892354355040000*cos(2*q2 + q3 + q5) + 204918069092352000*cos(q3 - 2*q4 + q5) - 688511307840972000*cos(q3 + 2*q4 + q5) - 2802173268057527600*sin(2*q2 + q3 + q4) - 654294339572379000*sin(q3 + q4 - q5) + 263215575638400000*sin(q3 - q4 + q5) + 71554218859200000*sin(2*q2 + q4 + q5) + 102545161890029100*sin(q3 + q4 - 2*q5) - 86518873621629900*sin(q3 + q4 + 2*q5) - 1294599914315400000*sin(2*q3 + q4 + q5) - 17375927152419000*sin(q3 + q4 - 3*q5) + 14845172097789000*sin(q3 + q4 + 3*q5) + 129816178829568000*sin(q3 + 3*q4 + q5) - 747401719680000000*sin(3*q3 + q4 + q5) - 826334928787500*sin(q3 + q4 - 4*q5) + 826334928787500*sin(q3 + q4 + 4*q5) - 8026910600940000*cos(q3 + q5) - 307377103638528000*cos(2*q2 + q3 - 2*q4 - q5) + 68897040635808000*cos(2*q2 + q3 + 2*q4 - q5) + 361307719080000000*cos(2*q2 - q3 - 2*q4 + q5) + 133818527969280000*cos(2*q2 + q3 - 2*q4 - 2*q5) + 133818527969280000*cos(2*q2 + q3 - 2*q4 + 2*q5) + 95940149868486000*cos(2*q2 + q3 + 2*q4 - 2*q5) + 77902768388214000*cos(2*q2 + q3 + 2*q4 + 2*q5) + 130574643375000000*cos(2*q2 - 2*q3 - 2*q4 + q5) + 94503391863767040*cos(2*q2 + 2*q3 - 2*q4 + q5) - 79191348804751590*cos(2*q2 + 2*q3 + 2*q4 + q5) + 2791786688460000*cos(2*q2 + q3 + 2*q4 - 3*q5) + 5060899180260000*cos(2*q2 + q3 + 2*q4 + 3*q5) - 576295999026132000*cos(2*q2 + 3*q3 + 2*q4 + q5) - 493936096500000*cos(2*q2 + q3 + 2*q4 - 4*q5) - 493936096500000*cos(2*q2 + q3 + 2*q4 + 4*q5) + 5810099146494720*cos(2*q2 + 2*q3 + 4*q4 + q5) - 388795443590400000*cos(2*q2 + 4*q3 + 2*q4 + q5) + 6299214635868000*cos(2*q2 + 3*q3 + 4*q4 + q5) + 6214471984668750*cos(2*q2 + 4*q3 + 4*q4 + q5) - 1452769072173234800*sin(q3 + q4) + 1695144023107956960*sin(q4 + q5) - 434655564841344000*sin(2*q2 + q3 - q4 - q5) + 249133906560000000*sin(2*q2 - q3 + q4 - q5) - 541171909059375000*sin(2*q2 - q3 - q4 + q5) + 49749541180416000*sin(2*q2 + q3 - q4 - 2*q5) - 49749541180416000*sin(2*q2 + q3 - q4 + 2*q5) - 270106914000000000*sin(2*q2 - 2*q3 - q4 + q5) - 659458095958310880*sin(2*q2 + 2*q3 + q4 - q5) + 198288207833210880*sin(2*q2 + 2*q3 - q4 + q5) - 23469448464000000*sin(2*q2 + q3 - q4 - 3*q5) + 23469448464000000*sin(2*q2 + q3 - q4 + 3*q5) - 64908089414784000*sin(2*q2 + q3 + 3*q4 - q5) + 70214520701733408*sin(2*q2 + 2*q3 + q4 - 2*q5) - 28961365078733472*sin(2*q2 + 2*q3 + q4 + 2*q5) + 703860871308672000*sin(2*q2 + 3*q3 + q4 - q5) - 43126889541120000*sin(2*q2 + q3 + 3*q4 - 2*q5) - 43126889541120000*sin(2*q2 + q3 + 3*q4 + 2*q5) + 7229221519877280*sin(2*q2 + 2*q3 + q4 - 3*q5) - 10730595571930080*sin(2*q2 + 2*q3 + q4 + 3*q5) + 98765956556688960*sin(2*q2 + 2*q3 + 3*q4 + q5) + 12437385295104000*sin(2*q2 + 3*q3 + q4 - 2*q5) - 12437385295104000*sin(2*q2 + 3*q3 + q4 + 2*q5) + 459578782924800000*sin(2*q2 + 4*q3 + q4 - q5) - 9387779385600000*sin(2*q2 + q3 + 3*q4 - 3*q5) + 9387779385600000*sin(2*q2 + q3 + 3*q4 + 3*q5) - 508114967976000*sin(2*q2 + 2*q3 + q4 - 4*q5) + 508114967976000*sin(2*q2 + 2*q3 + q4 + 4*q5) + 139078540684066500*sin(2*q2 + 3*q3 + 3*q4 + q5) + 100469397659400000*sin(2*q2 + 4*q3 + 3*q4 + q5) + 5029599035533917600*cos(q3) - 15333099750698400*cos(q5) + 353017946300006400*cos(2*q2 + q3 - 2*q4) + 195374268399248400*cos(2*q2 + q3 + 2*q4) - 11430579338640000*cos(2*q2 + q3 - q5) - 94478739098713200*cos(2*q2 + q3 - 2*q5) - 124541041565833200*cos(2*q2 + q3 + 2*q5) - 3782170647763200*cos(2*q2 + 2*q3 + q5) - 204918069092352000*cos(q3 - 2*q4 - q5) + 675423498059772000*cos(q3 + 2*q4 - q5) + 6892354355040000*cos(2*q2 + q3 - 3*q5) + 11430579338640000*cos(2*q2 + q3 + 3*q5) + 444337649817600000*cos(2*q2 - 2*q4 + q5) - 166626618681600000*cos(2*q2 + 2*q4 + q5) + 89212351979520000*cos(q3 - 2*q4 - 2*q5) + 89212351979520000*cos(q3 - 2*q4 + 2*q5) + 327858343534260000*cos(q3 + 2*q4 - 2*q5) + 297796041067140000*cos(q3 + 2*q4 + 2*q5) - 1975744386000000*cos(2*q2 + q3 - 4*q5) - 1975744386000000*cos(2*q2 + q3 + 4*q5) - 965614734321600000*cos(2*q3 + 2*q4 + q5) - 1397988830700000*cos(q3 + 2*q4 - 3*q5) + 14485798611900000*cos(q3 + 2*q4 + 3*q5) - 481743625440000000*cos(3*q3 + 2*q4 + q5) - 2469680482500000*cos(q3 + 2*q4 - 4*q5) - 2469680482500000*cos(q3 + 2*q4 + 4*q5) - 3775857455561867648*sin(q4) + 944482049133414400*sin(2*q2 + q3 - q4) + 572253033856000000*sin(2*q2 - q3 + q4) - 1498149960073735360*sin(2*q2 + 2*q3 + q4) - 263215575638400000*sin(q3 - q4 - q5) - 13758230207052800*sin(2*q2 + q3 + 3*q4) - 71554218859200000*sin(2*q2 + q4 - q5) - 31194357763800000*sin(2*q2 - q4 + q5) + 1616747092278707200*sin(2*q2 + 3*q3 + q4) + 37312155885312000*sin(q3 - q4 - 2*q5) - 37312155885312000*sin(q3 - q4 + 2*q5) + 7639726386600000*sin(2*q2 + q4 - 2*q5) - 19329093768600000*sin(2*q2 + q4 + 2*q5) + 1055638537748480000*sin(2*q2 + 4*q3 + q4) + 1294599914315400000*sin(2*q3 + q4 - q5) - 229789391462400000*sin(2*q3 - q4 + q5) - 14081669078400000*sin(q3 - q4 - 3*q5) + 14081669078400000*sin(q3 - q4 + 3*q5) - 129816178829568000*sin(q3 + 3*q4 - q5) - 7633557855000000*sin(2*q2 + q4 - 3*q5) + 7633557855000000*sin(2*q2 + q4 + 3*q5) - 13943965681800000*sin(2*q3 + q4 - 2*q5) - 67881605992200000*sin(2*q3 + q4 + 2*q5) + 747401719680000000*sin(3*q3 + q4 - q5) - 86253779082240000*sin(q3 + 3*q4 - 2*q5) - 86253779082240000*sin(q3 + 3*q4 + 2*q5) - 22900673565000000*sin(2*q3 + q4 - 3*q5) + 22900673565000000*sin(2*q3 + q4 + 3*q5) + 138200062354200000*sin(2*q3 + 3*q4 + q5) - 18775558771200000*sin(q3 + 3*q4 - 3*q5) + 18775558771200000*sin(q3 + 3*q4 + 3*q5) + 73537762505625000*sin(3*q3 + 3*q4 + q5) + 1232782761435769500*sin(2*q2 + q3 + q4 + q5) + 7646094127248401852)^(1/2));
%    -(2^(1/2)*(27516460414105600*cos(q3 + 3*q4) - 5888866708854080000*cos(2*q3 + q4) - 572253033856000000*cos(q3 - q4) - 5150277304704000000*cos(3*q3 + q4) + 541171909059375000*cos(2*q2 - q3 - q4 - q5) + 20956287886875000*cos(2*q2 - q3 - q4 - 2*q5) - 8282866618125000*cos(2*q2 - q3 - q4 + 2*q5) + 540213828000000000*cos(2*q2 - 2*q3 - q4 - q5) + 396576415666421760*cos(2*q2 + 2*q3 - q4 - q5) - 8276178796875000*cos(2*q2 - q3 - q4 - 3*q5) + 8276178796875000*cos(2*q2 - q3 - q4 + 3*q5) - 45886635629936640*cos(2*q2 + 2*q3 - q4 - 2*q5) + 45886635629936640*cos(2*q2 + 2*q3 - q4 + 2*q5) + 17317691854848000*cos(2*q2 + 2*q3 - q4 - 3*q5) - 17317691854848000*cos(2*q2 + 2*q3 - q4 + 3*q5) + 192863414377307520*cos(2*q2 + 2*q3 + 3*q4 - q5) + 139667883829911360*cos(2*q2 + 2*q3 + 3*q4 - 2*q5) + 136338643638267840*cos(2*q2 + 2*q3 + 3*q4 + 2*q5) + 413439489470254500*cos(2*q2 + 3*q3 + 3*q4 - q5) + 34919056932883200*cos(2*q2 + 2*q3 + 3*q4 - 3*q5) - 30250558196812800*cos(2*q2 + 2*q3 + 3*q4 + 3*q5) + 263805157393049250*cos(2*q2 + 3*q3 + 3*q4 - 2*q5) + 261098026497420750*cos(2*q2 + 3*q3 + 3*q4 + 2*q5) + 401877590637600000*cos(2*q2 + 4*q3 + 3*q4 - q5) + 508114967976000*cos(2*q2 + 2*q3 + 3*q4 - 4*q5) - 508114967976000*cos(2*q2 + 2*q3 + 3*q4 + 4*q5) + 54889940838397500*cos(2*q2 + 3*q3 + 3*q4 - 3*q5) - 51093808256452500*cos(2*q2 + 3*q3 + 3*q4 + 3*q5) + 233787347640000000*cos(2*q2 + 4*q3 + 3*q4 - 2*q5) + 233787347640000000*cos(2*q2 + 4*q3 + 3*q4 + 2*q5) + 413167464393750*cos(2*q2 + 3*q3 + 3*q4 - 4*q5) - 413167464393750*cos(2*q2 + 3*q3 + 3*q4 + 4*q5) + 40712308560000000*cos(2*q2 + 4*q3 + 3*q4 - 3*q5) - 40712308560000000*cos(2*q2 + 4*q3 + 3*q4 + 3*q5) + 7263190296986061200*sin(2*q2 + q3) + 235345297533337600*sin(q3 - 2*q4) + 822231539407213600*sin(q3 + 2*q4) - 10296023092740000*sin(q3 - q5) - 70107391443751200*sin(q3 - 2*q5) - 76119851937175200*sin(q3 + 2*q5) + 8026910600940000*sin(q3 - 3*q5) + 10296023092740000*sin(q3 + 3*q5) - 493936096500000*sin(q3 - 4*q5) - 493936096500000*sin(q3 + 4*q5) + 361307719080000000*sin(2*q2 - q3 - 2*q4 - q5) - 131081296500000000*sin(2*q2 - q3 - 2*q4 - 2*q5) - 131081296500000000*sin(2*q2 - q3 - 2*q4 + 2*q5) + 261149286750000000*sin(2*q2 - 2*q3 - 2*q4 - q5) - 189006783727534080*sin(2*q2 + 2*q3 - 2*q4 - q5) + 127716498108106380*sin(2*q2 + 2*q3 + 2*q4 - q5) - 85269720937500000*sin(2*q2 - 2*q3 - 2*q4 - 2*q5) - 85269720937500000*sin(2*q2 - 2*q3 - 2*q4 + 2*q5) + 82285275237580800*sin(2*q2 + 2*q3 - 2*q4 - 2*q5) + 82285275237580800*sin(2*q2 + 2*q3 - 2*q4 + 2*q5) + 235845517878338346*sin(2*q2 + 2*q3 + 2*q4 - 2*q5) + 165406186902402666*sin(2*q2 + 2*q3 + 2*q4 + 2*q5) + 1713182625340956000*sin(2*q2 + 3*q3 + 2*q4 - q5) + 18769510446883020*sin(2*q2 + 2*q3 + 2*q4 - 3*q5) + 11896689054513780*sin(2*q2 + 2*q3 + 2*q4 + 3*q5) - 11620198292989440*sin(2*q2 + 2*q3 + 4*q4 - q5) + 538227120396042000*sin(2*q2 + 3*q3 + 2*q4 - 2*q5) + 502152357435498000*sin(2*q2 + 3*q3 + 2*q4 + 2*q5) + 1555181774361600000*sin(2*q2 + 4*q3 + 2*q4 - q5) + 748031352071850*sin(2*q2 + 2*q3 + 2*q4 - 4*q5) + 748031352071850*sin(2*q2 + 2*q3 + 2*q4 + 4*q5) - 15003495465235200*sin(2*q2 + 2*q3 + 4*q4 - 2*q5) - 15003495465235200*sin(2*q2 + 2*q3 + 4*q4 + 2*q5) + 7852685868720000*sin(2*q2 + 3*q3 + 2*q4 - 3*q5) + 7852685868720000*sin(2*q2 + 3*q3 + 2*q4 + 3*q5) - 18897643907604000*sin(2*q2 + 3*q3 + 4*q4 - q5) + 386890301952000000*sin(2*q2 + 4*q3 + 2*q4 - 2*q5) + 386890301952000000*sin(2*q2 + 4*q3 + 2*q4 + 2*q5) - 6278767742016000*sin(2*q2 + 2*q3 + 4*q4 - 3*q5) + 6278767742016000*sin(2*q2 + 2*q3 + 4*q4 + 3*q5) - 24399817242570000*sin(2*q2 + 3*q3 + 4*q4 - 2*q5) - 24399817242570000*sin(2*q2 + 3*q3 + 4*q4 + 2*q5) - 24857887938675000*sin(2*q2 + 4*q3 + 4*q4 - q5) - 911166822720000*sin(2*q2 + 2*q3 + 4*q4 - 4*q5) - 911166822720000*sin(2*q2 + 2*q3 + 4*q4 + 4*q5) - 10211006213100000*sin(2*q2 + 3*q3 + 4*q4 - 3*q5) + 10211006213100000*sin(2*q2 + 3*q3 + 4*q4 + 3*q5) - 32446417205812500*sin(2*q2 + 4*q3 + 4*q4 - 2*q5) - 32446417205812500*sin(2*q2 + 4*q3 + 4*q4 + 2*q5) - 1481808289500000*sin(2*q2 + 3*q3 + 4*q4 - 4*q5) - 1481808289500000*sin(2*q2 + 3*q3 + 4*q4 + 4*q5) - 12300673584375000*sin(2*q2 + 4*q3 + 4*q4 - 3*q5) + 12300673584375000*sin(2*q2 + 4*q3 + 4*q4 + 3*q5) - 1606552354687500*sin(2*q2 + 4*q3 + 4*q4 - 4*q5) - 1606552354687500*sin(2*q2 + 4*q3 + 4*q4 + 4*q5) - 656825094627009000*cos(q3 + q4 + q5) - 1249392186595000000*cos(2*q2 - q3 - q4) - 1240854792800000000*cos(2*q2 - 2*q3 - q4) - 871145795906584576*cos(2*q2 + 2*q3 - q4) + 63675071524036224*cos(2*q2 + 2*q3 + 3*q4) - 459578782924800000*cos(2*q3 - q4 - q5) + 51770936820158400*cos(2*q2 + 3*q3 + 3*q4) - 4016247658080000*cos(2*q2 + 4*q3 + 3*q4) + 276400124708400000*cos(2*q3 + 3*q4 - q5) + 175340510730000000*cos(2*q3 + 3*q4 - 2*q5) + 175340510730000000*cos(2*q3 + 3*q4 + 2*q5) + 220613287516875000*cos(3*q3 + 3*q4 - q5) + 35623269990000000*cos(2*q3 + 3*q4 - 3*q5) - 35623269990000000*cos(2*q3 + 3*q4 + 3*q5) + 133070923321875000*cos(3*q3 + 3*q4 - 2*q5) + 133070923321875000*cos(3*q3 + 3*q4 + 2*q5) + 24828536390625000*cos(3*q3 + 3*q4 - 3*q5) - 24828536390625000*cos(3*q3 + 3*q4 + 3*q5) - 9852939583065600000*sin(2*q3) - 7102581190656000000*sin(3*q3) - 362523922404000000*sin(2*q2 - q3 - 2*q4) - 52432518600000000*sin(2*q2 - q3 - 2*q5) - 52432518600000000*sin(2*q2 - q3 + 2*q5) - 243079518400000000*sin(2*q2 - 2*q3 - 2*q4) + 217071427371925504*sin(2*q2 + 2*q3 - 2*q4) + 438536338768182720*sin(2*q2 + 2*q3 + 2*q4) - 11750186456870400*sin(2*q2 + 2*q3 - q5) - 131469808648502016*sin(2*q2 + 2*q3 - 2*q5) - 175834693607037696*sin(2*q2 + 2*q3 + 2*q5) + 1518435668338738800*sin(2*q2 + 3*q3 + 2*q4) + 9532529563768064*sin(2*q2 + 2*q3 + 4*q4) + 7564341295526400*sin(2*q2 + 2*q3 - 3*q5) + 11750186456870400*sin(2*q2 + 2*q3 + 3*q5) + 1205767251566080000*sin(2*q2 + 4*q3 + 2*q4) + 1919877796894200000*sin(2*q3 + 2*q4 - q5) - 1822333645440000*sin(2*q2 + 2*q3 - 4*q5) - 1822333645440000*sin(2*q2 + 2*q3 + 4*q5) + 15502519379852400*sin(2*q2 + 3*q3 + 4*q4) + 623204391074512500*sin(2*q3 + 2*q4 - 2*q5) + 597129945057112500*sin(2*q3 + 2*q4 + 2*q5) + 1445230876320000000*sin(3*q3 + 2*q4 - q5) + 26989924537705000*sin(2*q2 + 4*q3 + 4*q4) - 9084972426750000*sin(2*q3 + 2*q4 - 3*q5) + 20436644175750000*sin(2*q3 + 2*q4 + 3*q5) + 393243889500000000*sin(3*q3 + 2*q4 - 2*q5) + 393243889500000000*sin(3*q3 + 2*q4 + 2*q5) - 3748622160937500*sin(2*q3 + 2*q4 - 4*q5) - 3748622160937500*sin(2*q3 + 2*q4 + 4*q5) + 1228986628853824500*cos(2*q2 + q3 + q4 - q5) - 434655564841344000*cos(2*q2 + q3 - q4 + q5) - 249133906560000000*cos(2*q2 - q3 + q4 + q5) - 66932179328831850*cos(2*q2 + q3 + q4 - 2*q5) + 38232469791682650*cos(2*q2 + q3 + q4 + 2*q5) - 1325918940020727360*cos(2*q2 + 2*q3 + q4 + q5) + 344657733601500*cos(2*q2 + q3 + q4 - 3*q5) + 3451474848343500*cos(2*q2 + q3 + q4 + 3*q5) - 64908089414784000*cos(2*q2 + q3 + 3*q4 + q5) + 2111582613926016000*cos(2*q2 + 3*q3 + q4 + q5) + 688612440656250*cos(2*q2 + q3 + q4 - 4*q5) - 688612440656250*cos(2*q2 + q3 + q4 + 4*q5) + 1838315131699200000*cos(2*q2 + 4*q3 + q4 + q5) + 307377103638528000*sin(2*q2 + q3 - 2*q4 + q5) - 76749726504528000*sin(2*q2 + q3 + 2*q4 + q5) + 1055638537748480000*cos(2*q3 - q4) + 36287059501280000*cos(2*q3 + 3*q4) + 10496246199000000*cos(3*q3 + 3*q4) + 2505845877220000000*sin(2*q2 - q3) + 2566834188800000000*sin(2*q2 - 2*q3) + 4963773870401251584*sin(2*q2 + 2*q3) - 6481926188417433600*sin(2*q2 + 3*q3) - 4367391100764160000*sin(2*q2 + 4*q3) + 1766797471532185000*sin(2*q3 + 2*q4) + 241806438720000000*sin(2*q3 - 2*q5) + 241806438720000000*sin(2*q3 + 2*q5) + 1187933096616000000*sin(3*q3 + 2*q4) + 2802173268057527600*cos(2*q2 + q3 + q4) + 654294339572379000*cos(q3 + q4 - q5) - 263215575638400000*cos(q3 - q4 + q5) - 102545161890029100*cos(q3 + q4 - 2*q5) + 86518873621629900*cos(q3 + q4 + 2*q5) + 2589199828630800000*cos(2*q3 + q4 + q5) + 17375927152419000*cos(q3 + q4 - 3*q5) - 14845172097789000*cos(q3 + q4 + 3*q5) - 129816178829568000*cos(q3 + 3*q4 + q5) + 2242205159040000000*cos(3*q3 + q4 + q5) + 826334928787500*cos(q3 + q4 - 4*q5) - 826334928787500*cos(q3 + q4 + 4*q5) - 6892354355040000*sin(2*q2 + q3 + q5) + 204918069092352000*sin(q3 - 2*q4 + q5) - 688511307840972000*sin(q3 + 2*q4 + q5) + 1452769072173234800*cos(q3 + q4) + 434655564841344000*cos(2*q2 + q3 - q4 - q5) + 249133906560000000*cos(2*q2 - q3 + q4 - q5) - 541171909059375000*cos(2*q2 - q3 - q4 + q5) - 49749541180416000*cos(2*q2 + q3 - q4 - 2*q5) + 49749541180416000*cos(2*q2 + q3 - q4 + 2*q5) - 540213828000000000*cos(2*q2 - 2*q3 - q4 + q5) + 1318916191916621760*cos(2*q2 + 2*q3 + q4 - q5) - 396576415666421760*cos(2*q2 + 2*q3 - q4 + q5) + 23469448464000000*cos(2*q2 + q3 - q4 - 3*q5) - 23469448464000000*cos(2*q2 + q3 - q4 + 3*q5) + 64908089414784000*cos(2*q2 + q3 + 3*q4 - q5) - 140429041403466816*cos(2*q2 + 2*q3 + q4 - 2*q5) + 57922730157466944*cos(2*q2 + 2*q3 + q4 + 2*q5) - 2111582613926016000*cos(2*q2 + 3*q3 + q4 - q5) + 43126889541120000*cos(2*q2 + q3 + 3*q4 - 2*q5) + 43126889541120000*cos(2*q2 + q3 + 3*q4 + 2*q5) - 14458443039754560*cos(2*q2 + 2*q3 + q4 - 3*q5) + 21461191143860160*cos(2*q2 + 2*q3 + q4 + 3*q5) - 197531913113377920*cos(2*q2 + 2*q3 + 3*q4 + q5) - 37312155885312000*cos(2*q2 + 3*q3 + q4 - 2*q5) + 37312155885312000*cos(2*q2 + 3*q3 + q4 + 2*q5) - 1838315131699200000*cos(2*q2 + 4*q3 + q4 - q5) + 9387779385600000*cos(2*q2 + q3 + 3*q4 - 3*q5) - 9387779385600000*cos(2*q2 + q3 + 3*q4 + 3*q5) + 1016229935952000*cos(2*q2 + 2*q3 + q4 - 4*q5) - 1016229935952000*cos(2*q2 + 2*q3 + q4 + 4*q5) - 417235622052199500*cos(2*q2 + 3*q3 + 3*q4 + q5) - 401877590637600000*cos(2*q2 + 4*q3 + 3*q4 + q5) - 8026910600940000*sin(q3 + q5) - 307377103638528000*sin(2*q2 + q3 - 2*q4 - q5) + 68897040635808000*sin(2*q2 + q3 + 2*q4 - q5) - 361307719080000000*sin(2*q2 - q3 - 2*q4 + q5) + 133818527969280000*sin(2*q2 + q3 - 2*q4 - 2*q5) + 133818527969280000*sin(2*q2 + q3 - 2*q4 + 2*q5) + 95940149868486000*sin(2*q2 + q3 + 2*q4 - 2*q5) + 77902768388214000*sin(2*q2 + q3 + 2*q4 + 2*q5) - 261149286750000000*sin(2*q2 - 2*q3 - 2*q4 + q5) + 189006783727534080*sin(2*q2 + 2*q3 - 2*q4 + q5) - 158382697609503180*sin(2*q2 + 2*q3 + 2*q4 + q5) + 2791786688460000*sin(2*q2 + q3 + 2*q4 - 3*q5) + 5060899180260000*sin(2*q2 + q3 + 2*q4 + 3*q5) - 1728887997078396000*sin(2*q2 + 3*q3 + 2*q4 + q5) - 493936096500000*sin(2*q2 + q3 + 2*q4 - 4*q5) - 493936096500000*sin(2*q2 + q3 + 2*q4 + 4*q5) + 11620198292989440*sin(2*q2 + 2*q3 + 4*q4 + q5) - 1555181774361600000*sin(2*q2 + 4*q3 + 2*q4 + q5) + 18897643907604000*sin(2*q2 + 3*q3 + 4*q4 + q5) + 24857887938675000*sin(2*q2 + 4*q3 + 4*q4 + q5) - 944482049133414400*cos(2*q2 + q3 - q4) + 572253033856000000*cos(2*q2 - q3 + q4) + 2996299920147470720*cos(2*q2 + 2*q3 + q4) + 263215575638400000*cos(q3 - q4 - q5) + 13758230207052800*cos(2*q2 + q3 + 3*q4) - 4850241276836121600*cos(2*q2 + 3*q3 + q4) - 37312155885312000*cos(q3 - q4 - 2*q5) + 37312155885312000*cos(q3 - q4 + 2*q5) - 4222554150993920000*cos(2*q2 + 4*q3 + q4) - 2589199828630800000*cos(2*q3 + q4 - q5) + 459578782924800000*cos(2*q3 - q4 + q5) + 14081669078400000*cos(q3 - q4 - 3*q5) - 14081669078400000*cos(q3 - q4 + 3*q5) + 129816178829568000*cos(q3 + 3*q4 - q5) + 27887931363600000*cos(2*q3 + q4 - 2*q5) + 135763211984400000*cos(2*q3 + q4 + 2*q5) - 2242205159040000000*cos(3*q3 + q4 - q5) + 86253779082240000*cos(q3 + 3*q4 - 2*q5) + 86253779082240000*cos(q3 + 3*q4 + 2*q5) + 45801347130000000*cos(2*q3 + q4 - 3*q5) - 45801347130000000*cos(2*q3 + q4 + 3*q5) - 276400124708400000*cos(2*q3 + 3*q4 + q5) + 18775558771200000*cos(q3 + 3*q4 - 3*q5) - 18775558771200000*cos(q3 + 3*q4 + 3*q5) - 220613287516875000*cos(3*q3 + 3*q4 + q5) + 5029599035533917600*sin(q3) + 353017946300006400*sin(2*q2 + q3 - 2*q4) + 195374268399248400*sin(2*q2 + q3 + 2*q4) - 11430579338640000*sin(2*q2 + q3 - q5) - 94478739098713200*sin(2*q2 + q3 - 2*q5) - 124541041565833200*sin(2*q2 + q3 + 2*q5) - 7564341295526400*sin(2*q2 + 2*q3 + q5) - 204918069092352000*sin(q3 - 2*q4 - q5) + 675423498059772000*sin(q3 + 2*q4 - q5) + 6892354355040000*sin(2*q2 + q3 - 3*q5) + 11430579338640000*sin(2*q2 + q3 + 3*q5) + 89212351979520000*sin(q3 - 2*q4 - 2*q5) + 89212351979520000*sin(q3 - 2*q4 + 2*q5) + 327858343534260000*sin(q3 + 2*q4 - 2*q5) + 297796041067140000*sin(q3 + 2*q4 + 2*q5) - 1975744386000000*sin(2*q2 + q3 - 4*q5) - 1975744386000000*sin(2*q2 + q3 + 4*q5) - 1931229468643200000*sin(2*q3 + 2*q4 + q5) - 1397988830700000*sin(q3 + 2*q4 - 3*q5) + 14485798611900000*sin(q3 + 2*q4 + 3*q5) - 1445230876320000000*sin(3*q3 + 2*q4 + q5) - 2469680482500000*sin(q3 + 2*q4 - 4*q5) - 2469680482500000*sin(q3 + 2*q4 + 4*q5) - 1232782761435769500*cos(2*q2 + q3 + q4 + q5)))/(128*(7263190296986061200*cos(2*q2 + q3) + 235345297533337600*cos(q3 - 2*q4) + 822231539407213600*cos(q3 + 2*q4) - 10296023092740000*cos(q3 - q5) - 2222884258031250*cos(2*q2 + q5) - 70107391443751200*cos(q3 - 2*q5) - 76119851937175200*cos(q3 + 2*q5) + 8026910600940000*cos(q3 - 3*q5) + 10296023092740000*cos(q3 + 3*q5) - 445882949398656000*cos(2*q4 + q5) - 493936096500000*cos(q3 - 4*q5) - 493936096500000*cos(q3 + 4*q5) - 361307719080000000*cos(2*q2 - q3 - 2*q4 - q5) + 131081296500000000*cos(2*q2 - q3 - 2*q4 - 2*q5) + 131081296500000000*cos(2*q2 - q3 - 2*q4 + 2*q5) - 130574643375000000*cos(2*q2 - 2*q3 - 2*q4 - q5) - 94503391863767040*cos(2*q2 + 2*q3 - 2*q4 - q5) + 63858249054053190*cos(2*q2 + 2*q3 + 2*q4 - q5) + 42634860468750000*cos(2*q2 - 2*q3 - 2*q4 - 2*q5) + 42634860468750000*cos(2*q2 - 2*q3 - 2*q4 + 2*q5) + 41142637618790400*cos(2*q2 + 2*q3 - 2*q4 - 2*q5) + 41142637618790400*cos(2*q2 + 2*q3 - 2*q4 + 2*q5) + 117922758939169173*cos(2*q2 + 2*q3 + 2*q4 - 2*q5) + 82703093451201333*cos(2*q2 + 2*q3 + 2*q4 + 2*q5) + 571060875113652000*cos(2*q2 + 3*q3 + 2*q4 - q5) + 9384755223441510*cos(2*q2 + 2*q3 + 2*q4 - 3*q5) + 5948344527256890*cos(2*q2 + 2*q3 + 2*q4 + 3*q5) - 5810099146494720*cos(2*q2 + 2*q3 + 4*q4 - q5) + 179409040132014000*cos(2*q2 + 3*q3 + 2*q4 - 2*q5) + 167384119145166000*cos(2*q2 + 3*q3 + 2*q4 + 2*q5) + 388795443590400000*cos(2*q2 + 4*q3 + 2*q4 - q5) + 374015676035925*cos(2*q2 + 2*q3 + 2*q4 - 4*q5) + 374015676035925*cos(2*q2 + 2*q3 + 2*q4 + 4*q5) - 7501747732617600*cos(2*q2 + 2*q3 + 4*q4 - 2*q5) - 7501747732617600*cos(2*q2 + 2*q3 + 4*q4 + 2*q5) + 2617561956240000*cos(2*q2 + 3*q3 + 2*q4 - 3*q5) + 2617561956240000*cos(2*q2 + 3*q3 + 2*q4 + 3*q5) - 6299214635868000*cos(2*q2 + 3*q3 + 4*q4 - q5) + 96722575488000000*cos(2*q2 + 4*q3 + 2*q4 - 2*q5) + 96722575488000000*cos(2*q2 + 4*q3 + 2*q4 + 2*q5) - 3139383871008000*cos(2*q2 + 2*q3 + 4*q4 - 3*q5) + 3139383871008000*cos(2*q2 + 2*q3 + 4*q4 + 3*q5) - 8133272414190000*cos(2*q2 + 3*q3 + 4*q4 - 2*q5) - 8133272414190000*cos(2*q2 + 3*q3 + 4*q4 + 2*q5) - 6214471984668750*cos(2*q2 + 4*q3 + 4*q4 - q5) - 455583411360000*cos(2*q2 + 2*q3 + 4*q4 - 4*q5) - 455583411360000*cos(2*q2 + 2*q3 + 4*q4 + 4*q5) - 3403668737700000*cos(2*q2 + 3*q3 + 4*q4 - 3*q5) + 3403668737700000*cos(2*q2 + 3*q3 + 4*q4 + 3*q5) - 8111604301453125*cos(2*q2 + 4*q3 + 4*q4 - 2*q5) - 8111604301453125*cos(2*q2 + 4*q3 + 4*q4 + 2*q5) - 493936096500000*cos(2*q2 + 3*q3 + 4*q4 - 4*q5) - 493936096500000*cos(2*q2 + 3*q3 + 4*q4 + 4*q5) - 3075168396093750*cos(2*q2 + 4*q3 + 4*q4 - 3*q5) + 3075168396093750*cos(2*q2 + 4*q3 + 4*q4 + 3*q5) - 401638088671875*cos(2*q2 + 4*q3 + 4*q4 - 4*q5) - 401638088671875*cos(2*q2 + 4*q3 + 4*q4 + 4*q5) + 572253033856000000*sin(q3 - q4) - 158513188718920000*sin(2*q2 + q4) + 2944433354427040000*sin(2*q3 + q4) - 27516460414105600*sin(q3 + 3*q4) - 1693976898423939360*sin(q4 - q5) + 1716759101568000000*sin(3*q3 + q4) + 153879467142538368*sin(q4 - 2*q5) - 54179474609538432*sin(q4 + 2*q5) - 7896057578529120*sin(q4 - 3*q5) + 6728932894511520*sin(q4 + 3*q5) + 59868167177871360*sin(q5 - 3*q4) + 59868167177871360*sin(3*q4 + q5) - 762172451964000*sin(q4 - 4*q5) + 762172451964000*sin(q4 + 4*q5) + 541171909059375000*sin(2*q2 - q3 - q4 - q5) + 20956287886875000*sin(2*q2 - q3 - q4 - 2*q5) - 8282866618125000*sin(2*q2 - q3 - q4 + 2*q5) + 270106914000000000*sin(2*q2 - 2*q3 - q4 - q5) - 198288207833210880*sin(2*q2 + 2*q3 - q4 - q5) - 8276178796875000*sin(2*q2 - q3 - q4 - 3*q5) + 8276178796875000*sin(2*q2 - q3 - q4 + 3*q5) + 22943317814968320*sin(2*q2 + 2*q3 - q4 - 2*q5) - 22943317814968320*sin(2*q2 + 2*q3 - q4 + 2*q5) - 8658845927424000*sin(2*q2 + 2*q3 - q4 - 3*q5) + 8658845927424000*sin(2*q2 + 2*q3 - q4 + 3*q5) - 96431707188653760*sin(2*q2 + 2*q3 + 3*q4 - q5) - 69833941914955680*sin(2*q2 + 2*q3 + 3*q4 - 2*q5) - 68169321819133920*sin(2*q2 + 2*q3 + 3*q4 + 2*q5) - 137813163156751500*sin(2*q2 + 3*q3 + 3*q4 - q5) - 17459528466441600*sin(2*q2 + 2*q3 + 3*q4 - 3*q5) + 15125279098406400*sin(2*q2 + 2*q3 + 3*q4 + 3*q5) - 87935052464349750*sin(2*q2 + 3*q3 + 3*q4 - 2*q5) - 87032675499140250*sin(2*q2 + 3*q3 + 3*q4 + 2*q5) - 100469397659400000*sin(2*q2 + 4*q3 + 3*q4 - q5) - 254057483988000*sin(2*q2 + 2*q3 + 3*q4 - 4*q5) + 254057483988000*sin(2*q2 + 2*q3 + 3*q4 + 4*q5) - 18296646946132500*sin(2*q2 + 3*q3 + 3*q4 - 3*q5) + 17031269418817500*sin(2*q2 + 3*q3 + 3*q4 + 3*q5) - 58446836910000000*sin(2*q2 + 4*q3 + 3*q4 - 2*q5) - 58446836910000000*sin(2*q2 + 4*q3 + 3*q4 + 2*q5) - 137722488131250*sin(2*q2 + 3*q3 + 3*q4 - 4*q5) + 137722488131250*sin(2*q2 + 3*q3 + 3*q4 + 4*q5) - 10178077140000000*sin(2*q2 + 4*q3 + 3*q4 - 3*q5) + 10178077140000000*sin(2*q2 + 4*q3 + 3*q4 + 3*q5) + 656825094627009000*sin(q3 + q4 + q5) + 2484582864105156250*cos(2*q2) - 4926469791532800000*cos(2*q3) - 2367527063552000000*cos(3*q3) + 588766372249655040*cos(2*q4) - 427286086914756762*cos(2*q5) + 15333099750698400*cos(3*q5) + 1659198174791850*cos(4*q5) + 362523922404000000*cos(2*q2 - q3 - 2*q4) + 52432518600000000*cos(2*q2 - q3 - 2*q5) + 52432518600000000*cos(2*q2 - q3 + 2*q5) + 121539759200000000*cos(2*q2 - 2*q3 - 2*q4) + 108535713685962752*cos(2*q2 + 2*q3 - 2*q4) + 219268169384091360*cos(2*q2 + 2*q3 + 2*q4) - 5875093228435200*cos(2*q2 + 2*q3 - q5) - 65734904324251008*cos(2*q2 + 2*q3 - 2*q5) - 87917346803518848*cos(2*q2 + 2*q3 + 2*q5) + 506145222779579600*cos(2*q2 + 3*q3 + 2*q4) - 444337649817600000*cos(2*q2 - 2*q4 - q5) + 166626618681600000*cos(2*q2 + 2*q4 - q5) + 4766264781884032*cos(2*q2 + 2*q3 + 4*q4) + 3782170647763200*cos(2*q2 + 2*q3 - 3*q5) + 5875093228435200*cos(2*q2 + 2*q3 + 3*q5) + 181354829040000000*cos(2*q2 - 2*q4 - 2*q5) + 181354829040000000*cos(2*q2 - 2*q4 + 2*q5) + 60451609680000000*cos(2*q2 + 2*q4 - 2*q5) + 60451609680000000*cos(2*q2 + 2*q4 + 2*q5) + 301441812891520000*cos(2*q2 + 4*q3 + 2*q4) + 959938898447100000*cos(2*q3 + 2*q4 - q5) - 911166822720000*cos(2*q2 + 2*q3 - 4*q5) - 911166822720000*cos(2*q2 + 2*q3 + 4*q5) + 5167506459950800*cos(2*q2 + 3*q3 + 4*q4) + 311602195537256250*cos(2*q3 + 2*q4 - 2*q5) + 298564972528556250*cos(2*q3 + 2*q4 + 2*q5) + 481743625440000000*cos(3*q3 + 2*q4 - q5) + 6747481134426250*cos(2*q2 + 4*q3 + 4*q4) - 4542486213375000*cos(2*q3 + 2*q4 - 3*q5) + 10218322087875000*cos(2*q3 + 2*q4 + 3*q5) + 131081296500000000*cos(3*q3 + 2*q4 - 2*q5) + 131081296500000000*cos(3*q3 + 2*q4 + 2*q5) - 1874311080468750*cos(2*q3 + 2*q4 - 4*q5) - 1874311080468750*cos(2*q3 + 2*q4 + 4*q5) - 12689944096858112*sin(3*q4) - 1249392186595000000*sin(2*q2 - q3 - q4) - 620427396400000000*sin(2*q2 - 2*q3 - q4) + 435572897953292288*sin(2*q2 + 2*q3 - q4) + 31194357763800000*sin(2*q2 - q4 - q5) - 31837535762018112*sin(2*q2 + 2*q3 + 3*q4) + 46297913923800000*sin(2*q2 - q4 - 2*q5) - 34608546541800000*sin(2*q2 - q4 + 2*q5) + 229789391462400000*sin(2*q3 - q4 - q5) - 22900673565000000*sin(2*q2 - q4 - 3*q5) + 22900673565000000*sin(2*q2 - q4 + 3*q5) - 17256978940052800*sin(2*q2 + 3*q3 + 3*q4) + 1004061914520000*sin(2*q2 + 4*q3 + 3*q4) - 138200062354200000*sin(2*q3 + 3*q4 - q5) - 87670255365000000*sin(2*q3 + 3*q4 - 2*q5) - 87670255365000000*sin(2*q3 + 3*q4 + 2*q5) - 73537762505625000*sin(3*q3 + 3*q4 - q5) - 17811634995000000*sin(2*q3 + 3*q4 - 3*q5) + 17811634995000000*sin(2*q3 + 3*q4 + 3*q5) - 44356974440625000*sin(3*q3 + 3*q4 - 2*q5) - 44356974440625000*sin(3*q3 + 3*q4 + 2*q5) - 8276178796875000*sin(3*q3 + 3*q4 - 3*q5) + 8276178796875000*sin(3*q3 + 3*q4 + 3*q5) + 307377103638528000*cos(2*q2 + q3 - 2*q4 + q5) - 76749726504528000*cos(2*q2 + q3 + 2*q4 + q5) - 1228986628853824500*sin(2*q2 + q3 + q4 - q5) + 434655564841344000*sin(2*q2 + q3 - q4 + q5) - 249133906560000000*sin(2*q2 - q3 + q4 + q5) + 66932179328831850*sin(2*q2 + q3 + q4 - 2*q5) - 38232469791682650*sin(2*q2 + q3 + q4 + 2*q5) + 662959470010363680*sin(2*q2 + 2*q3 + q4 + q5) - 344657733601500*sin(2*q2 + q3 + q4 - 3*q5) - 3451474848343500*sin(2*q2 + q3 + q4 + 3*q5) + 64908089414784000*sin(2*q2 + q3 + 3*q4 + q5) - 703860871308672000*sin(2*q2 + 3*q3 + q4 + q5) - 688612440656250*sin(2*q2 + q3 + q4 - 4*q5) + 688612440656250*sin(2*q2 + q3 + q4 + 4*q5) - 459578782924800000*sin(2*q2 + 4*q3 + q4 + q5) - 2505845877220000000*cos(2*q2 - q3) - 1283417094400000000*cos(2*q2 - 2*q3) + 2481886935200625792*cos(2*q2 + 2*q3) - 2160642062805811200*cos(2*q2 + 3*q3) + 486134414554880000*cos(2*q2 - 2*q4) + 167187503038080000*cos(2*q2 + 2*q4) - 3452951616468750*cos(2*q2 - q5) - 1091847775191040000*cos(2*q2 + 4*q3) + 25886953145356875*cos(2*q2 - 2*q5) + 12849730136656875*cos(2*q2 + 2*q5) + 883398735766092500*cos(2*q3 + 2*q4) + 2222884258031250*cos(2*q2 - 3*q5) + 3452951616468750*cos(2*q2 + 3*q5) + 120903219360000000*cos(2*q3 - 2*q5) + 120903219360000000*cos(2*q3 + 2*q5) + 395977698872000000*cos(3*q3 + 2*q4) + 436225685522457600*cos(2*q4 - q5) - 1472672991796875*cos(2*q2 - 4*q5) - 1472672991796875*cos(2*q2 + 4*q5) + 241523670772581120*cos(2*q4 - 2*q5) + 219341228293313280*cos(2*q4 + 2*q5) - 1450135803916800*cos(2*q4 - 3*q5) + 11107399680115200*cos(2*q4 + 3*q5) - 1822333645440000*cos(2*q4 - 4*q5) - 1822333645440000*cos(2*q4 + 4*q5) - 112565280336880000*sin(2*q2 - q4) - 527819268874240000*sin(2*q3 - q4) - 18143529750640000*sin(2*q3 + 3*q4) - 3498748733000000*sin(3*q3 + 3*q4) - 39778213412044800*sin(3*q4 - 2*q5) - 39778213412044800*sin(3*q4 + 2*q5) - 8658845927424000*sin(3*q4 - 3*q5) + 8658845927424000*sin(3*q4 + 3*q5) - 6892354355040000*cos(2*q2 + q3 + q5) + 204918069092352000*cos(q3 - 2*q4 + q5) - 688511307840972000*cos(q3 + 2*q4 + q5) - 2802173268057527600*sin(2*q2 + q3 + q4) - 654294339572379000*sin(q3 + q4 - q5) + 263215575638400000*sin(q3 - q4 + q5) + 71554218859200000*sin(2*q2 + q4 + q5) + 102545161890029100*sin(q3 + q4 - 2*q5) - 86518873621629900*sin(q3 + q4 + 2*q5) - 1294599914315400000*sin(2*q3 + q4 + q5) - 17375927152419000*sin(q3 + q4 - 3*q5) + 14845172097789000*sin(q3 + q4 + 3*q5) + 129816178829568000*sin(q3 + 3*q4 + q5) - 747401719680000000*sin(3*q3 + q4 + q5) - 826334928787500*sin(q3 + q4 - 4*q5) + 826334928787500*sin(q3 + q4 + 4*q5) - 8026910600940000*cos(q3 + q5) - 307377103638528000*cos(2*q2 + q3 - 2*q4 - q5) + 68897040635808000*cos(2*q2 + q3 + 2*q4 - q5) + 361307719080000000*cos(2*q2 - q3 - 2*q4 + q5) + 133818527969280000*cos(2*q2 + q3 - 2*q4 - 2*q5) + 133818527969280000*cos(2*q2 + q3 - 2*q4 + 2*q5) + 95940149868486000*cos(2*q2 + q3 + 2*q4 - 2*q5) + 77902768388214000*cos(2*q2 + q3 + 2*q4 + 2*q5) + 130574643375000000*cos(2*q2 - 2*q3 - 2*q4 + q5) + 94503391863767040*cos(2*q2 + 2*q3 - 2*q4 + q5) - 79191348804751590*cos(2*q2 + 2*q3 + 2*q4 + q5) + 2791786688460000*cos(2*q2 + q3 + 2*q4 - 3*q5) + 5060899180260000*cos(2*q2 + q3 + 2*q4 + 3*q5) - 576295999026132000*cos(2*q2 + 3*q3 + 2*q4 + q5) - 493936096500000*cos(2*q2 + q3 + 2*q4 - 4*q5) - 493936096500000*cos(2*q2 + q3 + 2*q4 + 4*q5) + 5810099146494720*cos(2*q2 + 2*q3 + 4*q4 + q5) - 388795443590400000*cos(2*q2 + 4*q3 + 2*q4 + q5) + 6299214635868000*cos(2*q2 + 3*q3 + 4*q4 + q5) + 6214471984668750*cos(2*q2 + 4*q3 + 4*q4 + q5) - 1452769072173234800*sin(q3 + q4) + 1695144023107956960*sin(q4 + q5) - 434655564841344000*sin(2*q2 + q3 - q4 - q5) + 249133906560000000*sin(2*q2 - q3 + q4 - q5) - 541171909059375000*sin(2*q2 - q3 - q4 + q5) + 49749541180416000*sin(2*q2 + q3 - q4 - 2*q5) - 49749541180416000*sin(2*q2 + q3 - q4 + 2*q5) - 270106914000000000*sin(2*q2 - 2*q3 - q4 + q5) - 659458095958310880*sin(2*q2 + 2*q3 + q4 - q5) + 198288207833210880*sin(2*q2 + 2*q3 - q4 + q5) - 23469448464000000*sin(2*q2 + q3 - q4 - 3*q5) + 23469448464000000*sin(2*q2 + q3 - q4 + 3*q5) - 64908089414784000*sin(2*q2 + q3 + 3*q4 - q5) + 70214520701733408*sin(2*q2 + 2*q3 + q4 - 2*q5) - 28961365078733472*sin(2*q2 + 2*q3 + q4 + 2*q5) + 703860871308672000*sin(2*q2 + 3*q3 + q4 - q5) - 43126889541120000*sin(2*q2 + q3 + 3*q4 - 2*q5) - 43126889541120000*sin(2*q2 + q3 + 3*q4 + 2*q5) + 7229221519877280*sin(2*q2 + 2*q3 + q4 - 3*q5) - 10730595571930080*sin(2*q2 + 2*q3 + q4 + 3*q5) + 98765956556688960*sin(2*q2 + 2*q3 + 3*q4 + q5) + 12437385295104000*sin(2*q2 + 3*q3 + q4 - 2*q5) - 12437385295104000*sin(2*q2 + 3*q3 + q4 + 2*q5) + 459578782924800000*sin(2*q2 + 4*q3 + q4 - q5) - 9387779385600000*sin(2*q2 + q3 + 3*q4 - 3*q5) + 9387779385600000*sin(2*q2 + q3 + 3*q4 + 3*q5) - 508114967976000*sin(2*q2 + 2*q3 + q4 - 4*q5) + 508114967976000*sin(2*q2 + 2*q3 + q4 + 4*q5) + 139078540684066500*sin(2*q2 + 3*q3 + 3*q4 + q5) + 100469397659400000*sin(2*q2 + 4*q3 + 3*q4 + q5) + 5029599035533917600*cos(q3) - 15333099750698400*cos(q5) + 353017946300006400*cos(2*q2 + q3 - 2*q4) + 195374268399248400*cos(2*q2 + q3 + 2*q4) - 11430579338640000*cos(2*q2 + q3 - q5) - 94478739098713200*cos(2*q2 + q3 - 2*q5) - 124541041565833200*cos(2*q2 + q3 + 2*q5) - 3782170647763200*cos(2*q2 + 2*q3 + q5) - 204918069092352000*cos(q3 - 2*q4 - q5) + 675423498059772000*cos(q3 + 2*q4 - q5) + 6892354355040000*cos(2*q2 + q3 - 3*q5) + 11430579338640000*cos(2*q2 + q3 + 3*q5) + 444337649817600000*cos(2*q2 - 2*q4 + q5) - 166626618681600000*cos(2*q2 + 2*q4 + q5) + 89212351979520000*cos(q3 - 2*q4 - 2*q5) + 89212351979520000*cos(q3 - 2*q4 + 2*q5) + 327858343534260000*cos(q3 + 2*q4 - 2*q5) + 297796041067140000*cos(q3 + 2*q4 + 2*q5) - 1975744386000000*cos(2*q2 + q3 - 4*q5) - 1975744386000000*cos(2*q2 + q3 + 4*q5) - 965614734321600000*cos(2*q3 + 2*q4 + q5) - 1397988830700000*cos(q3 + 2*q4 - 3*q5) + 14485798611900000*cos(q3 + 2*q4 + 3*q5) - 481743625440000000*cos(3*q3 + 2*q4 + q5) - 2469680482500000*cos(q3 + 2*q4 - 4*q5) - 2469680482500000*cos(q3 + 2*q4 + 4*q5) - 3775857455561867648*sin(q4) + 944482049133414400*sin(2*q2 + q3 - q4) + 572253033856000000*sin(2*q2 - q3 + q4) - 1498149960073735360*sin(2*q2 + 2*q3 + q4) - 263215575638400000*sin(q3 - q4 - q5) - 13758230207052800*sin(2*q2 + q3 + 3*q4) - 71554218859200000*sin(2*q2 + q4 - q5) - 31194357763800000*sin(2*q2 - q4 + q5) + 1616747092278707200*sin(2*q2 + 3*q3 + q4) + 37312155885312000*sin(q3 - q4 - 2*q5) - 37312155885312000*sin(q3 - q4 + 2*q5) + 7639726386600000*sin(2*q2 + q4 - 2*q5) - 19329093768600000*sin(2*q2 + q4 + 2*q5) + 1055638537748480000*sin(2*q2 + 4*q3 + q4) + 1294599914315400000*sin(2*q3 + q4 - q5) - 229789391462400000*sin(2*q3 - q4 + q5) - 14081669078400000*sin(q3 - q4 - 3*q5) + 14081669078400000*sin(q3 - q4 + 3*q5) - 129816178829568000*sin(q3 + 3*q4 - q5) - 7633557855000000*sin(2*q2 + q4 - 3*q5) + 7633557855000000*sin(2*q2 + q4 + 3*q5) - 13943965681800000*sin(2*q3 + q4 - 2*q5) - 67881605992200000*sin(2*q3 + q4 + 2*q5) + 747401719680000000*sin(3*q3 + q4 - q5) - 86253779082240000*sin(q3 + 3*q4 - 2*q5) - 86253779082240000*sin(q3 + 3*q4 + 2*q5) - 22900673565000000*sin(2*q3 + q4 - 3*q5) + 22900673565000000*sin(2*q3 + q4 + 3*q5) + 138200062354200000*sin(2*q3 + 3*q4 + q5) - 18775558771200000*sin(q3 + 3*q4 - 3*q5) + 18775558771200000*sin(q3 + 3*q4 + 3*q5) + 73537762505625000*sin(3*q3 + 3*q4 + q5) + 1232782761435769500*sin(2*q2 + q3 + q4 + q5) + 7646094127248401852)^(1/2));
%    -(2^(1/2)*(572253033856000000*cos(q3 - q4) + 158513188718920000*cos(2*q2 + q4) - 2944433354427040000*cos(2*q3 + q4) + 82549381242316800*cos(q3 + 3*q4) + 1693976898423939360*cos(q4 - q5) - 1716759101568000000*cos(3*q3 + q4) - 153879467142538368*cos(q4 - 2*q5) + 54179474609538432*cos(q4 + 2*q5) + 7896057578529120*cos(q4 - 3*q5) - 6728932894511520*cos(q4 + 3*q5) + 179604501533614080*cos(q5 - 3*q4) - 179604501533614080*cos(3*q4 + q5) + 762172451964000*cos(q4 - 4*q5) - 762172451964000*cos(q4 + 4*q5) + 541171909059375000*cos(2*q2 - q3 - q4 - q5) + 20956287886875000*cos(2*q2 - q3 - q4 - 2*q5) - 8282866618125000*cos(2*q2 - q3 - q4 + 2*q5) + 270106914000000000*cos(2*q2 - 2*q3 - q4 - q5) - 198288207833210880*cos(2*q2 + 2*q3 - q4 - q5) - 8276178796875000*cos(2*q2 - q3 - q4 - 3*q5) + 8276178796875000*cos(2*q2 - q3 - q4 + 3*q5) + 22943317814968320*cos(2*q2 + 2*q3 - q4 - 2*q5) - 22943317814968320*cos(2*q2 + 2*q3 - q4 + 2*q5) - 8658845927424000*cos(2*q2 + 2*q3 - q4 - 3*q5) + 8658845927424000*cos(2*q2 + 2*q3 - q4 + 3*q5) + 289295121565961280*cos(2*q2 + 2*q3 + 3*q4 - q5) + 209501825744867040*cos(2*q2 + 2*q3 + 3*q4 - 2*q5) + 204507965457401760*cos(2*q2 + 2*q3 + 3*q4 + 2*q5) + 413439489470254500*cos(2*q2 + 3*q3 + 3*q4 - q5) + 52378585399324800*cos(2*q2 + 2*q3 + 3*q4 - 3*q5) - 45375837295219200*cos(2*q2 + 2*q3 + 3*q4 + 3*q5) + 263805157393049250*cos(2*q2 + 3*q3 + 3*q4 - 2*q5) + 261098026497420750*cos(2*q2 + 3*q3 + 3*q4 + 2*q5) + 301408192978200000*cos(2*q2 + 4*q3 + 3*q4 - q5) + 762172451964000*cos(2*q2 + 2*q3 + 3*q4 - 4*q5) - 762172451964000*cos(2*q2 + 2*q3 + 3*q4 + 4*q5) + 54889940838397500*cos(2*q2 + 3*q3 + 3*q4 - 3*q5) - 51093808256452500*cos(2*q2 + 3*q3 + 3*q4 + 3*q5) + 175340510730000000*cos(2*q2 + 4*q3 + 3*q4 - 2*q5) + 175340510730000000*cos(2*q2 + 4*q3 + 3*q4 + 2*q5) + 413167464393750*cos(2*q2 + 3*q3 + 3*q4 - 4*q5) - 413167464393750*cos(2*q2 + 3*q3 + 3*q4 + 4*q5) + 30534231420000000*cos(2*q2 + 4*q3 + 3*q4 - 3*q5) - 30534231420000000*cos(2*q2 + 4*q3 + 3*q4 + 3*q5) - 470690595066675200*sin(q3 - 2*q4) + 1644463078814427200*sin(q3 + 2*q4) - 891765898797312000*sin(2*q4 + q5) + 722615438160000000*sin(2*q2 - q3 - 2*q4 - q5) - 262162593000000000*sin(2*q2 - q3 - 2*q4 - 2*q5) - 262162593000000000*sin(2*q2 - q3 - 2*q4 + 2*q5) + 261149286750000000*sin(2*q2 - 2*q3 - 2*q4 - q5) + 189006783727534080*sin(2*q2 + 2*q3 - 2*q4 - q5) + 127716498108106380*sin(2*q2 + 2*q3 + 2*q4 - q5) - 85269720937500000*sin(2*q2 - 2*q3 - 2*q4 - 2*q5) - 85269720937500000*sin(2*q2 - 2*q3 - 2*q4 + 2*q5) - 82285275237580800*sin(2*q2 + 2*q3 - 2*q4 - 2*q5) - 82285275237580800*sin(2*q2 + 2*q3 - 2*q4 + 2*q5) + 235845517878338346*sin(2*q2 + 2*q3 + 2*q4 - 2*q5) + 165406186902402666*sin(2*q2 + 2*q3 + 2*q4 + 2*q5) + 1142121750227304000*sin(2*q2 + 3*q3 + 2*q4 - q5) + 18769510446883020*sin(2*q2 + 2*q3 + 2*q4 - 3*q5) + 11896689054513780*sin(2*q2 + 2*q3 + 2*q4 + 3*q5) - 23240396585978880*sin(2*q2 + 2*q3 + 4*q4 - q5) + 358818080264028000*sin(2*q2 + 3*q3 + 2*q4 - 2*q5) + 334768238290332000*sin(2*q2 + 3*q3 + 2*q4 + 2*q5) + 777590887180800000*sin(2*q2 + 4*q3 + 2*q4 - q5) + 748031352071850*sin(2*q2 + 2*q3 + 2*q4 - 4*q5) + 748031352071850*sin(2*q2 + 2*q3 + 2*q4 + 4*q5) - 30006990930470400*sin(2*q2 + 2*q3 + 4*q4 - 2*q5) - 30006990930470400*sin(2*q2 + 2*q3 + 4*q4 + 2*q5) + 5235123912480000*sin(2*q2 + 3*q3 + 2*q4 - 3*q5) + 5235123912480000*sin(2*q2 + 3*q3 + 2*q4 + 3*q5) - 25196858543472000*sin(2*q2 + 3*q3 + 4*q4 - q5) + 193445150976000000*sin(2*q2 + 4*q3 + 2*q4 - 2*q5) + 193445150976000000*sin(2*q2 + 4*q3 + 2*q4 + 2*q5) - 12557535484032000*sin(2*q2 + 2*q3 + 4*q4 - 3*q5) + 12557535484032000*sin(2*q2 + 2*q3 + 4*q4 + 3*q5) - 32533089656760000*sin(2*q2 + 3*q3 + 4*q4 - 2*q5) - 32533089656760000*sin(2*q2 + 3*q3 + 4*q4 + 2*q5) - 24857887938675000*sin(2*q2 + 4*q3 + 4*q4 - q5) - 1822333645440000*sin(2*q2 + 2*q3 + 4*q4 - 4*q5) - 1822333645440000*sin(2*q2 + 2*q3 + 4*q4 + 4*q5) - 13614674950800000*sin(2*q2 + 3*q3 + 4*q4 - 3*q5) + 13614674950800000*sin(2*q2 + 3*q3 + 4*q4 + 3*q5) - 32446417205812500*sin(2*q2 + 4*q3 + 4*q4 - 2*q5) - 32446417205812500*sin(2*q2 + 4*q3 + 4*q4 + 2*q5) - 1975744386000000*sin(2*q2 + 3*q3 + 4*q4 - 4*q5) - 1975744386000000*sin(2*q2 + 3*q3 + 4*q4 + 4*q5) - 12300673584375000*sin(2*q2 + 4*q3 + 4*q4 - 3*q5) + 12300673584375000*sin(2*q2 + 4*q3 + 4*q4 + 3*q5) - 1606552354687500*sin(2*q2 + 4*q3 + 4*q4 - 4*q5) - 1606552354687500*sin(2*q2 + 4*q3 + 4*q4 + 4*q5) - 656825094627009000*cos(q3 + q4 + q5) + 38069832290574336*cos(3*q4) - 1249392186595000000*cos(2*q2 - q3 - q4) - 620427396400000000*cos(2*q2 - 2*q3 - q4) + 435572897953292288*cos(2*q2 + 2*q3 - q4) + 31194357763800000*cos(2*q2 - q4 - q5) + 95512607286054336*cos(2*q2 + 2*q3 + 3*q4) + 46297913923800000*cos(2*q2 - q4 - 2*q5) - 34608546541800000*cos(2*q2 - q4 + 2*q5) + 229789391462400000*cos(2*q3 - q4 - q5) - 22900673565000000*cos(2*q2 - q4 - 3*q5) + 22900673565000000*cos(2*q2 - q4 + 3*q5) + 51770936820158400*cos(2*q2 + 3*q3 + 3*q4) - 3012185743560000*cos(2*q2 + 4*q3 + 3*q4) + 414600187062600000*cos(2*q3 + 3*q4 - q5) + 263010766095000000*cos(2*q3 + 3*q4 - 2*q5) + 263010766095000000*cos(2*q3 + 3*q4 + 2*q5) + 220613287516875000*cos(3*q3 + 3*q4 - q5) + 53434904985000000*cos(2*q3 + 3*q4 - 3*q5) - 53434904985000000*cos(2*q3 + 3*q4 + 3*q5) + 133070923321875000*cos(3*q3 + 3*q4 - 2*q5) + 133070923321875000*cos(3*q3 + 3*q4 + 2*q5) + 24828536390625000*cos(3*q3 + 3*q4 - 3*q5) - 24828536390625000*cos(3*q3 + 3*q4 + 3*q5) + 1177532744499310080*sin(2*q4) - 725047844808000000*sin(2*q2 - q3 - 2*q4) - 243079518400000000*sin(2*q2 - 2*q3 - 2*q4) - 217071427371925504*sin(2*q2 + 2*q3 - 2*q4) + 438536338768182720*sin(2*q2 + 2*q3 + 2*q4) + 1012290445559159200*sin(2*q2 + 3*q3 + 2*q4) + 888675299635200000*sin(2*q2 - 2*q4 - q5) + 333253237363200000*sin(2*q2 + 2*q4 - q5) + 19065059127536128*sin(2*q2 + 2*q3 + 4*q4) - 362709658080000000*sin(2*q2 - 2*q4 - 2*q5) - 362709658080000000*sin(2*q2 - 2*q4 + 2*q5) + 120903219360000000*sin(2*q2 + 2*q4 - 2*q5) + 120903219360000000*sin(2*q2 + 2*q4 + 2*q5) + 602883625783040000*sin(2*q2 + 4*q3 + 2*q4) + 1919877796894200000*sin(2*q3 + 2*q4 - q5) + 20670025839803200*sin(2*q2 + 3*q3 + 4*q4) + 623204391074512500*sin(2*q3 + 2*q4 - 2*q5) + 597129945057112500*sin(2*q3 + 2*q4 + 2*q5) + 963487250880000000*sin(3*q3 + 2*q4 - q5) + 26989924537705000*sin(2*q2 + 4*q3 + 4*q4) - 9084972426750000*sin(2*q3 + 2*q4 - 3*q5) + 20436644175750000*sin(2*q3 + 2*q4 + 3*q5) + 262162593000000000*sin(3*q3 + 2*q4 - 2*q5) + 262162593000000000*sin(3*q3 + 2*q4 + 2*q5) - 3748622160937500*sin(2*q3 + 2*q4 - 4*q5) - 3748622160937500*sin(2*q3 + 2*q4 + 4*q5) + 1228986628853824500*cos(2*q2 + q3 + q4 - q5) + 434655564841344000*cos(2*q2 + q3 - q4 + q5) + 249133906560000000*cos(2*q2 - q3 + q4 + q5) - 66932179328831850*cos(2*q2 + q3 + q4 - 2*q5) + 38232469791682650*cos(2*q2 + q3 + q4 + 2*q5) - 662959470010363680*cos(2*q2 + 2*q3 + q4 + q5) + 344657733601500*cos(2*q2 + q3 + q4 - 3*q5) + 3451474848343500*cos(2*q2 + q3 + q4 + 3*q5) - 194724268244352000*cos(2*q2 + q3 + 3*q4 + q5) + 703860871308672000*cos(2*q2 + 3*q3 + q4 + q5) + 688612440656250*cos(2*q2 + q3 + q4 - 4*q5) - 688612440656250*cos(2*q2 + q3 + q4 + 4*q5) + 459578782924800000*cos(2*q2 + 4*q3 + q4 + q5) - 614754207277056000*sin(2*q2 + q3 - 2*q4 + q5) - 153499453009056000*sin(2*q2 + q3 + 2*q4 + q5) - 112565280336880000*cos(2*q2 - q4) - 527819268874240000*cos(2*q3 - q4) + 54430589251920000*cos(2*q3 + 3*q4) + 10496246199000000*cos(3*q3 + 3*q4) + 119334640236134400*cos(3*q4 - 2*q5) + 119334640236134400*cos(3*q4 + 2*q5) + 25976537782272000*cos(3*q4 - 3*q5) - 25976537782272000*cos(3*q4 + 3*q5) - 972268829109760000*sin(2*q2 - 2*q4) + 334375006076160000*sin(2*q2 + 2*q4) + 1766797471532185000*sin(2*q3 + 2*q4) + 791955397744000000*sin(3*q3 + 2*q4) + 872451371044915200*sin(2*q4 - q5) + 483047341545162240*sin(2*q4 - 2*q5) + 438682456586626560*sin(2*q4 + 2*q5) - 2900271607833600*sin(2*q4 - 3*q5) + 22214799360230400*sin(2*q4 + 3*q5) - 3644667290880000*sin(2*q4 - 4*q5) - 3644667290880000*sin(2*q4 + 4*q5) + 2802173268057527600*cos(2*q2 + q3 + q4) + 654294339572379000*cos(q3 + q4 - q5) + 263215575638400000*cos(q3 - q4 + q5) - 71554218859200000*cos(2*q2 + q4 + q5) - 102545161890029100*cos(q3 + q4 - 2*q5) + 86518873621629900*cos(q3 + q4 + 2*q5) + 1294599914315400000*cos(2*q3 + q4 + q5) + 17375927152419000*cos(q3 + q4 - 3*q5) - 14845172097789000*cos(q3 + q4 + 3*q5) - 389448536488704000*cos(q3 + 3*q4 + q5) + 747401719680000000*cos(3*q3 + q4 + q5) + 826334928787500*cos(q3 + q4 - 4*q5) - 826334928787500*cos(q3 + q4 + 4*q5) - 409836138184704000*sin(q3 - 2*q4 + q5) - 1377022615681944000*sin(q3 + 2*q4 + q5) + 1452769072173234800*cos(q3 + q4) - 1695144023107956960*cos(q4 + q5) - 434655564841344000*cos(2*q2 + q3 - q4 - q5) - 249133906560000000*cos(2*q2 - q3 + q4 - q5) - 541171909059375000*cos(2*q2 - q3 - q4 + q5) + 49749541180416000*cos(2*q2 + q3 - q4 - 2*q5) - 49749541180416000*cos(2*q2 + q3 - q4 + 2*q5) - 270106914000000000*cos(2*q2 - 2*q3 - q4 + q5) + 659458095958310880*cos(2*q2 + 2*q3 + q4 - q5) + 198288207833210880*cos(2*q2 + 2*q3 - q4 + q5) - 23469448464000000*cos(2*q2 + q3 - q4 - 3*q5) + 23469448464000000*cos(2*q2 + q3 - q4 + 3*q5) + 194724268244352000*cos(2*q2 + q3 + 3*q4 - q5) - 70214520701733408*cos(2*q2 + 2*q3 + q4 - 2*q5) + 28961365078733472*cos(2*q2 + 2*q3 + q4 + 2*q5) - 703860871308672000*cos(2*q2 + 3*q3 + q4 - q5) + 129380668623360000*cos(2*q2 + q3 + 3*q4 - 2*q5) + 129380668623360000*cos(2*q2 + q3 + 3*q4 + 2*q5) - 7229221519877280*cos(2*q2 + 2*q3 + q4 - 3*q5) + 10730595571930080*cos(2*q2 + 2*q3 + q4 + 3*q5) - 296297869670066880*cos(2*q2 + 2*q3 + 3*q4 + q5) - 12437385295104000*cos(2*q2 + 3*q3 + q4 - 2*q5) + 12437385295104000*cos(2*q2 + 3*q3 + q4 + 2*q5) - 459578782924800000*cos(2*q2 + 4*q3 + q4 - q5) + 28163338156800000*cos(2*q2 + q3 + 3*q4 - 3*q5) - 28163338156800000*cos(2*q2 + q3 + 3*q4 + 3*q5) + 508114967976000*cos(2*q2 + 2*q3 + q4 - 4*q5) - 508114967976000*cos(2*q2 + 2*q3 + q4 + 4*q5) - 417235622052199500*cos(2*q2 + 3*q3 + 3*q4 + q5) - 301408192978200000*cos(2*q2 + 4*q3 + 3*q4 + q5) + 614754207277056000*sin(2*q2 + q3 - 2*q4 - q5) + 137794081271616000*sin(2*q2 + q3 + 2*q4 - q5) - 722615438160000000*sin(2*q2 - q3 - 2*q4 + q5) - 267637055938560000*sin(2*q2 + q3 - 2*q4 - 2*q5) - 267637055938560000*sin(2*q2 + q3 - 2*q4 + 2*q5) + 191880299736972000*sin(2*q2 + q3 + 2*q4 - 2*q5) + 155805536776428000*sin(2*q2 + q3 + 2*q4 + 2*q5) - 261149286750000000*sin(2*q2 - 2*q3 - 2*q4 + q5) - 189006783727534080*sin(2*q2 + 2*q3 - 2*q4 + q5) - 158382697609503180*sin(2*q2 + 2*q3 + 2*q4 + q5) + 5583573376920000*sin(2*q2 + q3 + 2*q4 - 3*q5) + 10121798360520000*sin(2*q2 + q3 + 2*q4 + 3*q5) - 1152591998052264000*sin(2*q2 + 3*q3 + 2*q4 + q5) - 987872193000000*sin(2*q2 + q3 + 2*q4 - 4*q5) - 987872193000000*sin(2*q2 + q3 + 2*q4 + 4*q5) + 23240396585978880*sin(2*q2 + 2*q3 + 4*q4 + q5) - 777590887180800000*sin(2*q2 + 4*q3 + 2*q4 + q5) + 25196858543472000*sin(2*q2 + 3*q3 + 4*q4 + q5) + 24857887938675000*sin(2*q2 + 4*q3 + 4*q4 + q5) + 3775857455561867648*cos(q4) + 944482049133414400*cos(2*q2 + q3 - q4) - 572253033856000000*cos(2*q2 - q3 + q4) + 1498149960073735360*cos(2*q2 + 2*q3 + q4) - 263215575638400000*cos(q3 - q4 - q5) + 41274690621158400*cos(2*q2 + q3 + 3*q4) + 71554218859200000*cos(2*q2 + q4 - q5) - 31194357763800000*cos(2*q2 - q4 + q5) - 1616747092278707200*cos(2*q2 + 3*q3 + q4) + 37312155885312000*cos(q3 - q4 - 2*q5) - 37312155885312000*cos(q3 - q4 + 2*q5) - 7639726386600000*cos(2*q2 + q4 - 2*q5) + 19329093768600000*cos(2*q2 + q4 + 2*q5) - 1055638537748480000*cos(2*q2 + 4*q3 + q4) - 1294599914315400000*cos(2*q3 + q4 - q5) - 229789391462400000*cos(2*q3 - q4 + q5) - 14081669078400000*cos(q3 - q4 - 3*q5) + 14081669078400000*cos(q3 - q4 + 3*q5) + 389448536488704000*cos(q3 + 3*q4 - q5) + 7633557855000000*cos(2*q2 + q4 - 3*q5) - 7633557855000000*cos(2*q2 + q4 + 3*q5) + 13943965681800000*cos(2*q3 + q4 - 2*q5) + 67881605992200000*cos(2*q3 + q4 + 2*q5) - 747401719680000000*cos(3*q3 + q4 - q5) + 258761337246720000*cos(q3 + 3*q4 - 2*q5) + 258761337246720000*cos(q3 + 3*q4 + 2*q5) + 22900673565000000*cos(2*q3 + q4 - 3*q5) - 22900673565000000*cos(2*q3 + q4 + 3*q5) - 414600187062600000*cos(2*q3 + 3*q4 + q5) + 56326676313600000*cos(q3 + 3*q4 - 3*q5) - 56326676313600000*cos(q3 + 3*q4 + 3*q5) - 220613287516875000*cos(3*q3 + 3*q4 + q5) - 706035892600012800*sin(2*q2 + q3 - 2*q4) + 390748536798496800*sin(2*q2 + q3 + 2*q4) + 409836138184704000*sin(q3 - 2*q4 - q5) + 1350846996119544000*sin(q3 + 2*q4 - q5) - 888675299635200000*sin(2*q2 - 2*q4 + q5) - 333253237363200000*sin(2*q2 + 2*q4 + q5) - 178424703959040000*sin(q3 - 2*q4 - 2*q5) - 178424703959040000*sin(q3 - 2*q4 + 2*q5) + 655716687068520000*sin(q3 + 2*q4 - 2*q5) + 595592082134280000*sin(q3 + 2*q4 + 2*q5) - 1931229468643200000*sin(2*q3 + 2*q4 + q5) - 2795977661400000*sin(q3 + 2*q4 - 3*q5) + 28971597223800000*sin(q3 + 2*q4 + 3*q5) - 963487250880000000*sin(3*q3 + 2*q4 + q5) - 4939360965000000*sin(q3 + 2*q4 - 4*q5) - 4939360965000000*sin(q3 + 2*q4 + 4*q5) - 1232782761435769500*cos(2*q2 + q3 + q4 + q5)))/(128*(7263190296986061200*cos(2*q2 + q3) + 235345297533337600*cos(q3 - 2*q4) + 822231539407213600*cos(q3 + 2*q4) - 10296023092740000*cos(q3 - q5) - 2222884258031250*cos(2*q2 + q5) - 70107391443751200*cos(q3 - 2*q5) - 76119851937175200*cos(q3 + 2*q5) + 8026910600940000*cos(q3 - 3*q5) + 10296023092740000*cos(q3 + 3*q5) - 445882949398656000*cos(2*q4 + q5) - 493936096500000*cos(q3 - 4*q5) - 493936096500000*cos(q3 + 4*q5) - 361307719080000000*cos(2*q2 - q3 - 2*q4 - q5) + 131081296500000000*cos(2*q2 - q3 - 2*q4 - 2*q5) + 131081296500000000*cos(2*q2 - q3 - 2*q4 + 2*q5) - 130574643375000000*cos(2*q2 - 2*q3 - 2*q4 - q5) - 94503391863767040*cos(2*q2 + 2*q3 - 2*q4 - q5) + 63858249054053190*cos(2*q2 + 2*q3 + 2*q4 - q5) + 42634860468750000*cos(2*q2 - 2*q3 - 2*q4 - 2*q5) + 42634860468750000*cos(2*q2 - 2*q3 - 2*q4 + 2*q5) + 41142637618790400*cos(2*q2 + 2*q3 - 2*q4 - 2*q5) + 41142637618790400*cos(2*q2 + 2*q3 - 2*q4 + 2*q5) + 117922758939169173*cos(2*q2 + 2*q3 + 2*q4 - 2*q5) + 82703093451201333*cos(2*q2 + 2*q3 + 2*q4 + 2*q5) + 571060875113652000*cos(2*q2 + 3*q3 + 2*q4 - q5) + 9384755223441510*cos(2*q2 + 2*q3 + 2*q4 - 3*q5) + 5948344527256890*cos(2*q2 + 2*q3 + 2*q4 + 3*q5) - 5810099146494720*cos(2*q2 + 2*q3 + 4*q4 - q5) + 179409040132014000*cos(2*q2 + 3*q3 + 2*q4 - 2*q5) + 167384119145166000*cos(2*q2 + 3*q3 + 2*q4 + 2*q5) + 388795443590400000*cos(2*q2 + 4*q3 + 2*q4 - q5) + 374015676035925*cos(2*q2 + 2*q3 + 2*q4 - 4*q5) + 374015676035925*cos(2*q2 + 2*q3 + 2*q4 + 4*q5) - 7501747732617600*cos(2*q2 + 2*q3 + 4*q4 - 2*q5) - 7501747732617600*cos(2*q2 + 2*q3 + 4*q4 + 2*q5) + 2617561956240000*cos(2*q2 + 3*q3 + 2*q4 - 3*q5) + 2617561956240000*cos(2*q2 + 3*q3 + 2*q4 + 3*q5) - 6299214635868000*cos(2*q2 + 3*q3 + 4*q4 - q5) + 96722575488000000*cos(2*q2 + 4*q3 + 2*q4 - 2*q5) + 96722575488000000*cos(2*q2 + 4*q3 + 2*q4 + 2*q5) - 3139383871008000*cos(2*q2 + 2*q3 + 4*q4 - 3*q5) + 3139383871008000*cos(2*q2 + 2*q3 + 4*q4 + 3*q5) - 8133272414190000*cos(2*q2 + 3*q3 + 4*q4 - 2*q5) - 8133272414190000*cos(2*q2 + 3*q3 + 4*q4 + 2*q5) - 6214471984668750*cos(2*q2 + 4*q3 + 4*q4 - q5) - 455583411360000*cos(2*q2 + 2*q3 + 4*q4 - 4*q5) - 455583411360000*cos(2*q2 + 2*q3 + 4*q4 + 4*q5) - 3403668737700000*cos(2*q2 + 3*q3 + 4*q4 - 3*q5) + 3403668737700000*cos(2*q2 + 3*q3 + 4*q4 + 3*q5) - 8111604301453125*cos(2*q2 + 4*q3 + 4*q4 - 2*q5) - 8111604301453125*cos(2*q2 + 4*q3 + 4*q4 + 2*q5) - 493936096500000*cos(2*q2 + 3*q3 + 4*q4 - 4*q5) - 493936096500000*cos(2*q2 + 3*q3 + 4*q4 + 4*q5) - 3075168396093750*cos(2*q2 + 4*q3 + 4*q4 - 3*q5) + 3075168396093750*cos(2*q2 + 4*q3 + 4*q4 + 3*q5) - 401638088671875*cos(2*q2 + 4*q3 + 4*q4 - 4*q5) - 401638088671875*cos(2*q2 + 4*q3 + 4*q4 + 4*q5) + 572253033856000000*sin(q3 - q4) - 158513188718920000*sin(2*q2 + q4) + 2944433354427040000*sin(2*q3 + q4) - 27516460414105600*sin(q3 + 3*q4) - 1693976898423939360*sin(q4 - q5) + 1716759101568000000*sin(3*q3 + q4) + 153879467142538368*sin(q4 - 2*q5) - 54179474609538432*sin(q4 + 2*q5) - 7896057578529120*sin(q4 - 3*q5) + 6728932894511520*sin(q4 + 3*q5) + 59868167177871360*sin(q5 - 3*q4) + 59868167177871360*sin(3*q4 + q5) - 762172451964000*sin(q4 - 4*q5) + 762172451964000*sin(q4 + 4*q5) + 541171909059375000*sin(2*q2 - q3 - q4 - q5) + 20956287886875000*sin(2*q2 - q3 - q4 - 2*q5) - 8282866618125000*sin(2*q2 - q3 - q4 + 2*q5) + 270106914000000000*sin(2*q2 - 2*q3 - q4 - q5) - 198288207833210880*sin(2*q2 + 2*q3 - q4 - q5) - 8276178796875000*sin(2*q2 - q3 - q4 - 3*q5) + 8276178796875000*sin(2*q2 - q3 - q4 + 3*q5) + 22943317814968320*sin(2*q2 + 2*q3 - q4 - 2*q5) - 22943317814968320*sin(2*q2 + 2*q3 - q4 + 2*q5) - 8658845927424000*sin(2*q2 + 2*q3 - q4 - 3*q5) + 8658845927424000*sin(2*q2 + 2*q3 - q4 + 3*q5) - 96431707188653760*sin(2*q2 + 2*q3 + 3*q4 - q5) - 69833941914955680*sin(2*q2 + 2*q3 + 3*q4 - 2*q5) - 68169321819133920*sin(2*q2 + 2*q3 + 3*q4 + 2*q5) - 137813163156751500*sin(2*q2 + 3*q3 + 3*q4 - q5) - 17459528466441600*sin(2*q2 + 2*q3 + 3*q4 - 3*q5) + 15125279098406400*sin(2*q2 + 2*q3 + 3*q4 + 3*q5) - 87935052464349750*sin(2*q2 + 3*q3 + 3*q4 - 2*q5) - 87032675499140250*sin(2*q2 + 3*q3 + 3*q4 + 2*q5) - 100469397659400000*sin(2*q2 + 4*q3 + 3*q4 - q5) - 254057483988000*sin(2*q2 + 2*q3 + 3*q4 - 4*q5) + 254057483988000*sin(2*q2 + 2*q3 + 3*q4 + 4*q5) - 18296646946132500*sin(2*q2 + 3*q3 + 3*q4 - 3*q5) + 17031269418817500*sin(2*q2 + 3*q3 + 3*q4 + 3*q5) - 58446836910000000*sin(2*q2 + 4*q3 + 3*q4 - 2*q5) - 58446836910000000*sin(2*q2 + 4*q3 + 3*q4 + 2*q5) - 137722488131250*sin(2*q2 + 3*q3 + 3*q4 - 4*q5) + 137722488131250*sin(2*q2 + 3*q3 + 3*q4 + 4*q5) - 10178077140000000*sin(2*q2 + 4*q3 + 3*q4 - 3*q5) + 10178077140000000*sin(2*q2 + 4*q3 + 3*q4 + 3*q5) + 656825094627009000*sin(q3 + q4 + q5) + 2484582864105156250*cos(2*q2) - 4926469791532800000*cos(2*q3) - 2367527063552000000*cos(3*q3) + 588766372249655040*cos(2*q4) - 427286086914756762*cos(2*q5) + 15333099750698400*cos(3*q5) + 1659198174791850*cos(4*q5) + 362523922404000000*cos(2*q2 - q3 - 2*q4) + 52432518600000000*cos(2*q2 - q3 - 2*q5) + 52432518600000000*cos(2*q2 - q3 + 2*q5) + 121539759200000000*cos(2*q2 - 2*q3 - 2*q4) + 108535713685962752*cos(2*q2 + 2*q3 - 2*q4) + 219268169384091360*cos(2*q2 + 2*q3 + 2*q4) - 5875093228435200*cos(2*q2 + 2*q3 - q5) - 65734904324251008*cos(2*q2 + 2*q3 - 2*q5) - 87917346803518848*cos(2*q2 + 2*q3 + 2*q5) + 506145222779579600*cos(2*q2 + 3*q3 + 2*q4) - 444337649817600000*cos(2*q2 - 2*q4 - q5) + 166626618681600000*cos(2*q2 + 2*q4 - q5) + 4766264781884032*cos(2*q2 + 2*q3 + 4*q4) + 3782170647763200*cos(2*q2 + 2*q3 - 3*q5) + 5875093228435200*cos(2*q2 + 2*q3 + 3*q5) + 181354829040000000*cos(2*q2 - 2*q4 - 2*q5) + 181354829040000000*cos(2*q2 - 2*q4 + 2*q5) + 60451609680000000*cos(2*q2 + 2*q4 - 2*q5) + 60451609680000000*cos(2*q2 + 2*q4 + 2*q5) + 301441812891520000*cos(2*q2 + 4*q3 + 2*q4) + 959938898447100000*cos(2*q3 + 2*q4 - q5) - 911166822720000*cos(2*q2 + 2*q3 - 4*q5) - 911166822720000*cos(2*q2 + 2*q3 + 4*q5) + 5167506459950800*cos(2*q2 + 3*q3 + 4*q4) + 311602195537256250*cos(2*q3 + 2*q4 - 2*q5) + 298564972528556250*cos(2*q3 + 2*q4 + 2*q5) + 481743625440000000*cos(3*q3 + 2*q4 - q5) + 6747481134426250*cos(2*q2 + 4*q3 + 4*q4) - 4542486213375000*cos(2*q3 + 2*q4 - 3*q5) + 10218322087875000*cos(2*q3 + 2*q4 + 3*q5) + 131081296500000000*cos(3*q3 + 2*q4 - 2*q5) + 131081296500000000*cos(3*q3 + 2*q4 + 2*q5) - 1874311080468750*cos(2*q3 + 2*q4 - 4*q5) - 1874311080468750*cos(2*q3 + 2*q4 + 4*q5) - 12689944096858112*sin(3*q4) - 1249392186595000000*sin(2*q2 - q3 - q4) - 620427396400000000*sin(2*q2 - 2*q3 - q4) + 435572897953292288*sin(2*q2 + 2*q3 - q4) + 31194357763800000*sin(2*q2 - q4 - q5) - 31837535762018112*sin(2*q2 + 2*q3 + 3*q4) + 46297913923800000*sin(2*q2 - q4 - 2*q5) - 34608546541800000*sin(2*q2 - q4 + 2*q5) + 229789391462400000*sin(2*q3 - q4 - q5) - 22900673565000000*sin(2*q2 - q4 - 3*q5) + 22900673565000000*sin(2*q2 - q4 + 3*q5) - 17256978940052800*sin(2*q2 + 3*q3 + 3*q4) + 1004061914520000*sin(2*q2 + 4*q3 + 3*q4) - 138200062354200000*sin(2*q3 + 3*q4 - q5) - 87670255365000000*sin(2*q3 + 3*q4 - 2*q5) - 87670255365000000*sin(2*q3 + 3*q4 + 2*q5) - 73537762505625000*sin(3*q3 + 3*q4 - q5) - 17811634995000000*sin(2*q3 + 3*q4 - 3*q5) + 17811634995000000*sin(2*q3 + 3*q4 + 3*q5) - 44356974440625000*sin(3*q3 + 3*q4 - 2*q5) - 44356974440625000*sin(3*q3 + 3*q4 + 2*q5) - 8276178796875000*sin(3*q3 + 3*q4 - 3*q5) + 8276178796875000*sin(3*q3 + 3*q4 + 3*q5) + 307377103638528000*cos(2*q2 + q3 - 2*q4 + q5) - 76749726504528000*cos(2*q2 + q3 + 2*q4 + q5) - 1228986628853824500*sin(2*q2 + q3 + q4 - q5) + 434655564841344000*sin(2*q2 + q3 - q4 + q5) - 249133906560000000*sin(2*q2 - q3 + q4 + q5) + 66932179328831850*sin(2*q2 + q3 + q4 - 2*q5) - 38232469791682650*sin(2*q2 + q3 + q4 + 2*q5) + 662959470010363680*sin(2*q2 + 2*q3 + q4 + q5) - 344657733601500*sin(2*q2 + q3 + q4 - 3*q5) - 3451474848343500*sin(2*q2 + q3 + q4 + 3*q5) + 64908089414784000*sin(2*q2 + q3 + 3*q4 + q5) - 703860871308672000*sin(2*q2 + 3*q3 + q4 + q5) - 688612440656250*sin(2*q2 + q3 + q4 - 4*q5) + 688612440656250*sin(2*q2 + q3 + q4 + 4*q5) - 459578782924800000*sin(2*q2 + 4*q3 + q4 + q5) - 2505845877220000000*cos(2*q2 - q3) - 1283417094400000000*cos(2*q2 - 2*q3) + 2481886935200625792*cos(2*q2 + 2*q3) - 2160642062805811200*cos(2*q2 + 3*q3) + 486134414554880000*cos(2*q2 - 2*q4) + 167187503038080000*cos(2*q2 + 2*q4) - 3452951616468750*cos(2*q2 - q5) - 1091847775191040000*cos(2*q2 + 4*q3) + 25886953145356875*cos(2*q2 - 2*q5) + 12849730136656875*cos(2*q2 + 2*q5) + 883398735766092500*cos(2*q3 + 2*q4) + 2222884258031250*cos(2*q2 - 3*q5) + 3452951616468750*cos(2*q2 + 3*q5) + 120903219360000000*cos(2*q3 - 2*q5) + 120903219360000000*cos(2*q3 + 2*q5) + 395977698872000000*cos(3*q3 + 2*q4) + 436225685522457600*cos(2*q4 - q5) - 1472672991796875*cos(2*q2 - 4*q5) - 1472672991796875*cos(2*q2 + 4*q5) + 241523670772581120*cos(2*q4 - 2*q5) + 219341228293313280*cos(2*q4 + 2*q5) - 1450135803916800*cos(2*q4 - 3*q5) + 11107399680115200*cos(2*q4 + 3*q5) - 1822333645440000*cos(2*q4 - 4*q5) - 1822333645440000*cos(2*q4 + 4*q5) - 112565280336880000*sin(2*q2 - q4) - 527819268874240000*sin(2*q3 - q4) - 18143529750640000*sin(2*q3 + 3*q4) - 3498748733000000*sin(3*q3 + 3*q4) - 39778213412044800*sin(3*q4 - 2*q5) - 39778213412044800*sin(3*q4 + 2*q5) - 8658845927424000*sin(3*q4 - 3*q5) + 8658845927424000*sin(3*q4 + 3*q5) - 6892354355040000*cos(2*q2 + q3 + q5) + 204918069092352000*cos(q3 - 2*q4 + q5) - 688511307840972000*cos(q3 + 2*q4 + q5) - 2802173268057527600*sin(2*q2 + q3 + q4) - 654294339572379000*sin(q3 + q4 - q5) + 263215575638400000*sin(q3 - q4 + q5) + 71554218859200000*sin(2*q2 + q4 + q5) + 102545161890029100*sin(q3 + q4 - 2*q5) - 86518873621629900*sin(q3 + q4 + 2*q5) - 1294599914315400000*sin(2*q3 + q4 + q5) - 17375927152419000*sin(q3 + q4 - 3*q5) + 14845172097789000*sin(q3 + q4 + 3*q5) + 129816178829568000*sin(q3 + 3*q4 + q5) - 747401719680000000*sin(3*q3 + q4 + q5) - 826334928787500*sin(q3 + q4 - 4*q5) + 826334928787500*sin(q3 + q4 + 4*q5) - 8026910600940000*cos(q3 + q5) - 307377103638528000*cos(2*q2 + q3 - 2*q4 - q5) + 68897040635808000*cos(2*q2 + q3 + 2*q4 - q5) + 361307719080000000*cos(2*q2 - q3 - 2*q4 + q5) + 133818527969280000*cos(2*q2 + q3 - 2*q4 - 2*q5) + 133818527969280000*cos(2*q2 + q3 - 2*q4 + 2*q5) + 95940149868486000*cos(2*q2 + q3 + 2*q4 - 2*q5) + 77902768388214000*cos(2*q2 + q3 + 2*q4 + 2*q5) + 130574643375000000*cos(2*q2 - 2*q3 - 2*q4 + q5) + 94503391863767040*cos(2*q2 + 2*q3 - 2*q4 + q5) - 79191348804751590*cos(2*q2 + 2*q3 + 2*q4 + q5) + 2791786688460000*cos(2*q2 + q3 + 2*q4 - 3*q5) + 5060899180260000*cos(2*q2 + q3 + 2*q4 + 3*q5) - 576295999026132000*cos(2*q2 + 3*q3 + 2*q4 + q5) - 493936096500000*cos(2*q2 + q3 + 2*q4 - 4*q5) - 493936096500000*cos(2*q2 + q3 + 2*q4 + 4*q5) + 5810099146494720*cos(2*q2 + 2*q3 + 4*q4 + q5) - 388795443590400000*cos(2*q2 + 4*q3 + 2*q4 + q5) + 6299214635868000*cos(2*q2 + 3*q3 + 4*q4 + q5) + 6214471984668750*cos(2*q2 + 4*q3 + 4*q4 + q5) - 1452769072173234800*sin(q3 + q4) + 1695144023107956960*sin(q4 + q5) - 434655564841344000*sin(2*q2 + q3 - q4 - q5) + 249133906560000000*sin(2*q2 - q3 + q4 - q5) - 541171909059375000*sin(2*q2 - q3 - q4 + q5) + 49749541180416000*sin(2*q2 + q3 - q4 - 2*q5) - 49749541180416000*sin(2*q2 + q3 - q4 + 2*q5) - 270106914000000000*sin(2*q2 - 2*q3 - q4 + q5) - 659458095958310880*sin(2*q2 + 2*q3 + q4 - q5) + 198288207833210880*sin(2*q2 + 2*q3 - q4 + q5) - 23469448464000000*sin(2*q2 + q3 - q4 - 3*q5) + 23469448464000000*sin(2*q2 + q3 - q4 + 3*q5) - 64908089414784000*sin(2*q2 + q3 + 3*q4 - q5) + 70214520701733408*sin(2*q2 + 2*q3 + q4 - 2*q5) - 28961365078733472*sin(2*q2 + 2*q3 + q4 + 2*q5) + 703860871308672000*sin(2*q2 + 3*q3 + q4 - q5) - 43126889541120000*sin(2*q2 + q3 + 3*q4 - 2*q5) - 43126889541120000*sin(2*q2 + q3 + 3*q4 + 2*q5) + 7229221519877280*sin(2*q2 + 2*q3 + q4 - 3*q5) - 10730595571930080*sin(2*q2 + 2*q3 + q4 + 3*q5) + 98765956556688960*sin(2*q2 + 2*q3 + 3*q4 + q5) + 12437385295104000*sin(2*q2 + 3*q3 + q4 - 2*q5) - 12437385295104000*sin(2*q2 + 3*q3 + q4 + 2*q5) + 459578782924800000*sin(2*q2 + 4*q3 + q4 - q5) - 9387779385600000*sin(2*q2 + q3 + 3*q4 - 3*q5) + 9387779385600000*sin(2*q2 + q3 + 3*q4 + 3*q5) - 508114967976000*sin(2*q2 + 2*q3 + q4 - 4*q5) + 508114967976000*sin(2*q2 + 2*q3 + q4 + 4*q5) + 139078540684066500*sin(2*q2 + 3*q3 + 3*q4 + q5) + 100469397659400000*sin(2*q2 + 4*q3 + 3*q4 + q5) + 5029599035533917600*cos(q3) - 15333099750698400*cos(q5) + 353017946300006400*cos(2*q2 + q3 - 2*q4) + 195374268399248400*cos(2*q2 + q3 + 2*q4) - 11430579338640000*cos(2*q2 + q3 - q5) - 94478739098713200*cos(2*q2 + q3 - 2*q5) - 124541041565833200*cos(2*q2 + q3 + 2*q5) - 3782170647763200*cos(2*q2 + 2*q3 + q5) - 204918069092352000*cos(q3 - 2*q4 - q5) + 675423498059772000*cos(q3 + 2*q4 - q5) + 6892354355040000*cos(2*q2 + q3 - 3*q5) + 11430579338640000*cos(2*q2 + q3 + 3*q5) + 444337649817600000*cos(2*q2 - 2*q4 + q5) - 166626618681600000*cos(2*q2 + 2*q4 + q5) + 89212351979520000*cos(q3 - 2*q4 - 2*q5) + 89212351979520000*cos(q3 - 2*q4 + 2*q5) + 327858343534260000*cos(q3 + 2*q4 - 2*q5) + 297796041067140000*cos(q3 + 2*q4 + 2*q5) - 1975744386000000*cos(2*q2 + q3 - 4*q5) - 1975744386000000*cos(2*q2 + q3 + 4*q5) - 965614734321600000*cos(2*q3 + 2*q4 + q5) - 1397988830700000*cos(q3 + 2*q4 - 3*q5) + 14485798611900000*cos(q3 + 2*q4 + 3*q5) - 481743625440000000*cos(3*q3 + 2*q4 + q5) - 2469680482500000*cos(q3 + 2*q4 - 4*q5) - 2469680482500000*cos(q3 + 2*q4 + 4*q5) - 3775857455561867648*sin(q4) + 944482049133414400*sin(2*q2 + q3 - q4) + 572253033856000000*sin(2*q2 - q3 + q4) - 1498149960073735360*sin(2*q2 + 2*q3 + q4) - 263215575638400000*sin(q3 - q4 - q5) - 13758230207052800*sin(2*q2 + q3 + 3*q4) - 71554218859200000*sin(2*q2 + q4 - q5) - 31194357763800000*sin(2*q2 - q4 + q5) + 1616747092278707200*sin(2*q2 + 3*q3 + q4) + 37312155885312000*sin(q3 - q4 - 2*q5) - 37312155885312000*sin(q3 - q4 + 2*q5) + 7639726386600000*sin(2*q2 + q4 - 2*q5) - 19329093768600000*sin(2*q2 + q4 + 2*q5) + 1055638537748480000*sin(2*q2 + 4*q3 + q4) + 1294599914315400000*sin(2*q3 + q4 - q5) - 229789391462400000*sin(2*q3 - q4 + q5) - 14081669078400000*sin(q3 - q4 - 3*q5) + 14081669078400000*sin(q3 - q4 + 3*q5) - 129816178829568000*sin(q3 + 3*q4 - q5) - 7633557855000000*sin(2*q2 + q4 - 3*q5) + 7633557855000000*sin(2*q2 + q4 + 3*q5) - 13943965681800000*sin(2*q3 + q4 - 2*q5) - 67881605992200000*sin(2*q3 + q4 + 2*q5) + 747401719680000000*sin(3*q3 + q4 - q5) - 86253779082240000*sin(q3 + 3*q4 - 2*q5) - 86253779082240000*sin(q3 + 3*q4 + 2*q5) - 22900673565000000*sin(2*q3 + q4 - 3*q5) + 22900673565000000*sin(2*q3 + q4 + 3*q5) + 138200062354200000*sin(2*q3 + 3*q4 + q5) - 18775558771200000*sin(q3 + 3*q4 - 3*q5) + 18775558771200000*sin(q3 + 3*q4 + 3*q5) + 73537762505625000*sin(3*q3 + 3*q4 + q5) + 1232782761435769500*sin(2*q2 + q3 + q4 + q5) + 7646094127248401852)^(1/2));
%    (2^(1/2)*(1693976898423939360*cos(q4 - q5) - 307758934285076736*cos(q4 - 2*q5) - 108358949219076864*cos(q4 + 2*q5) + 23688172735587360*cos(q4 - 3*q5) + 20186798683534560*cos(q4 + 3*q5) + 59868167177871360*cos(q5 - 3*q4) + 59868167177871360*cos(3*q4 + q5) + 3048689807856000*cos(q4 - 4*q5) + 3048689807856000*cos(q4 + 4*q5) - 541171909059375000*cos(2*q2 - q3 - q4 - q5) - 41912575773750000*cos(2*q2 - q3 - q4 - 2*q5) - 16565733236250000*cos(2*q2 - q3 - q4 + 2*q5) - 270106914000000000*cos(2*q2 - 2*q3 - q4 - q5) + 198288207833210880*cos(2*q2 + 2*q3 - q4 - q5) + 24828536390625000*cos(2*q2 - q3 - q4 - 3*q5) + 24828536390625000*cos(2*q2 - q3 - q4 + 3*q5) - 45886635629936640*cos(2*q2 + 2*q3 - q4 - 2*q5) - 45886635629936640*cos(2*q2 + 2*q3 - q4 + 2*q5) + 25976537782272000*cos(2*q2 + 2*q3 - q4 - 3*q5) + 25976537782272000*cos(2*q2 + 2*q3 - q4 + 3*q5) + 96431707188653760*cos(2*q2 + 2*q3 + 3*q4 - q5) + 139667883829911360*cos(2*q2 + 2*q3 + 3*q4 - 2*q5) - 136338643638267840*cos(2*q2 + 2*q3 + 3*q4 + 2*q5) + 137813163156751500*cos(2*q2 + 3*q3 + 3*q4 - q5) + 52378585399324800*cos(2*q2 + 2*q3 + 3*q4 - 3*q5) + 45375837295219200*cos(2*q2 + 2*q3 + 3*q4 + 3*q5) + 175870104928699500*cos(2*q2 + 3*q3 + 3*q4 - 2*q5) - 174065350998280500*cos(2*q2 + 3*q3 + 3*q4 + 2*q5) + 100469397659400000*cos(2*q2 + 4*q3 + 3*q4 - q5) + 1016229935952000*cos(2*q2 + 2*q3 + 3*q4 - 4*q5) + 1016229935952000*cos(2*q2 + 2*q3 + 3*q4 + 4*q5) + 54889940838397500*cos(2*q2 + 3*q3 + 3*q4 - 3*q5) + 51093808256452500*cos(2*q2 + 3*q3 + 3*q4 + 3*q5) + 116893673820000000*cos(2*q2 + 4*q3 + 3*q4 - 2*q5) - 116893673820000000*cos(2*q2 + 4*q3 + 3*q4 + 2*q5) + 550889952525000*cos(2*q2 + 3*q3 + 3*q4 - 4*q5) + 550889952525000*cos(2*q2 + 3*q3 + 3*q4 + 4*q5) + 30534231420000000*cos(2*q2 + 4*q3 + 3*q4 - 3*q5) + 30534231420000000*cos(2*q2 + 4*q3 + 3*q4 + 3*q5) - 10296023092740000*sin(q3 - q5) + 2222884258031250*sin(2*q2 + q5) - 140214782887502400*sin(q3 - 2*q5) + 152239703874350400*sin(q3 + 2*q5) + 24080731802820000*sin(q3 - 3*q5) - 30888069278220000*sin(q3 + 3*q5) + 445882949398656000*sin(2*q4 + q5) - 1975744386000000*sin(q3 - 4*q5) + 1975744386000000*sin(q3 + 4*q5) - 361307719080000000*sin(2*q2 - q3 - 2*q4 - q5) + 262162593000000000*sin(2*q2 - q3 - 2*q4 - 2*q5) - 262162593000000000*sin(2*q2 - q3 - 2*q4 + 2*q5) - 130574643375000000*sin(2*q2 - 2*q3 - 2*q4 - q5) - 94503391863767040*sin(2*q2 + 2*q3 - 2*q4 - q5) + 63858249054053190*sin(2*q2 + 2*q3 + 2*q4 - q5) + 85269720937500000*sin(2*q2 - 2*q3 - 2*q4 - 2*q5) - 85269720937500000*sin(2*q2 - 2*q3 - 2*q4 + 2*q5) + 82285275237580800*sin(2*q2 + 2*q3 - 2*q4 - 2*q5) - 82285275237580800*sin(2*q2 + 2*q3 - 2*q4 + 2*q5) + 235845517878338346*sin(2*q2 + 2*q3 + 2*q4 - 2*q5) - 165406186902402666*sin(2*q2 + 2*q3 + 2*q4 + 2*q5) + 571060875113652000*sin(2*q2 + 3*q3 + 2*q4 - q5) + 28154265670324530*sin(2*q2 + 2*q3 + 2*q4 - 3*q5) - 17845033581770670*sin(2*q2 + 2*q3 + 2*q4 + 3*q5) - 5810099146494720*sin(2*q2 + 2*q3 + 4*q4 - q5) + 358818080264028000*sin(2*q2 + 3*q3 + 2*q4 - 2*q5) - 334768238290332000*sin(2*q2 + 3*q3 + 2*q4 + 2*q5) + 388795443590400000*sin(2*q2 + 4*q3 + 2*q4 - q5) + 1496062704143700*sin(2*q2 + 2*q3 + 2*q4 - 4*q5) - 1496062704143700*sin(2*q2 + 2*q3 + 2*q4 + 4*q5) - 15003495465235200*sin(2*q2 + 2*q3 + 4*q4 - 2*q5) + 15003495465235200*sin(2*q2 + 2*q3 + 4*q4 + 2*q5) + 7852685868720000*sin(2*q2 + 3*q3 + 2*q4 - 3*q5) - 7852685868720000*sin(2*q2 + 3*q3 + 2*q4 + 3*q5) - 6299214635868000*sin(2*q2 + 3*q3 + 4*q4 - q5) + 193445150976000000*sin(2*q2 + 4*q3 + 2*q4 - 2*q5) - 193445150976000000*sin(2*q2 + 4*q3 + 2*q4 + 2*q5) - 9418151613024000*sin(2*q2 + 2*q3 + 4*q4 - 3*q5) - 9418151613024000*sin(2*q2 + 2*q3 + 4*q4 + 3*q5) - 16266544828380000*sin(2*q2 + 3*q3 + 4*q4 - 2*q5) + 16266544828380000*sin(2*q2 + 3*q3 + 4*q4 + 2*q5) - 6214471984668750*sin(2*q2 + 4*q3 + 4*q4 - q5) - 1822333645440000*sin(2*q2 + 2*q3 + 4*q4 - 4*q5) + 1822333645440000*sin(2*q2 + 2*q3 + 4*q4 + 4*q5) - 10211006213100000*sin(2*q2 + 3*q3 + 4*q4 - 3*q5) - 10211006213100000*sin(2*q2 + 3*q3 + 4*q4 + 3*q5) - 16223208602906250*sin(2*q2 + 4*q3 + 4*q4 - 2*q5) + 16223208602906250*sin(2*q2 + 4*q3 + 4*q4 + 2*q5) - 1975744386000000*sin(2*q2 + 3*q3 + 4*q4 - 4*q5) + 1975744386000000*sin(2*q2 + 3*q3 + 4*q4 + 4*q5) - 9225505188281250*sin(2*q2 + 4*q3 + 4*q4 - 3*q5) - 9225505188281250*sin(2*q2 + 4*q3 + 4*q4 + 3*q5) - 1606552354687500*sin(2*q2 + 4*q3 + 4*q4 - 4*q5) + 1606552354687500*sin(2*q2 + 4*q3 + 4*q4 + 4*q5) + 656825094627009000*cos(q3 + q4 + q5) - 31194357763800000*cos(2*q2 - q4 - q5) - 92595827847600000*cos(2*q2 - q4 - 2*q5) - 69217093083600000*cos(2*q2 - q4 + 2*q5) - 229789391462400000*cos(2*q3 - q4 - q5) + 68702020695000000*cos(2*q2 - q4 - 3*q5) + 68702020695000000*cos(2*q2 - q4 + 3*q5) + 138200062354200000*cos(2*q3 + 3*q4 - q5) + 175340510730000000*cos(2*q3 + 3*q4 - 2*q5) - 175340510730000000*cos(2*q3 + 3*q4 + 2*q5) + 73537762505625000*cos(3*q3 + 3*q4 - q5) + 53434904985000000*cos(2*q3 + 3*q4 - 3*q5) + 53434904985000000*cos(2*q3 + 3*q4 + 3*q5) + 88713948881250000*cos(3*q3 + 3*q4 - 2*q5) - 88713948881250000*cos(3*q3 + 3*q4 + 2*q5) + 24828536390625000*cos(3*q3 + 3*q4 - 3*q5) + 24828536390625000*cos(3*q3 + 3*q4 + 3*q5) + 854572173829513524*sin(2*q5) - 45999299252095200*sin(3*q5) - 6636792699167400*sin(4*q5) + 104865037200000000*sin(2*q2 - q3 - 2*q5) - 104865037200000000*sin(2*q2 - q3 + 2*q5) - 5875093228435200*sin(2*q2 + 2*q3 - q5) - 131469808648502016*sin(2*q2 + 2*q3 - 2*q5) + 175834693607037696*sin(2*q2 + 2*q3 + 2*q5) - 444337649817600000*sin(2*q2 - 2*q4 - q5) + 166626618681600000*sin(2*q2 + 2*q4 - q5) + 11346511943289600*sin(2*q2 + 2*q3 - 3*q5) - 17625279685305600*sin(2*q2 + 2*q3 + 3*q5) + 362709658080000000*sin(2*q2 - 2*q4 - 2*q5) - 362709658080000000*sin(2*q2 - 2*q4 + 2*q5) + 120903219360000000*sin(2*q2 + 2*q4 - 2*q5) - 120903219360000000*sin(2*q2 + 2*q4 + 2*q5) + 959938898447100000*sin(2*q3 + 2*q4 - q5) - 3644667290880000*sin(2*q2 + 2*q3 - 4*q5) + 3644667290880000*sin(2*q2 + 2*q3 + 4*q5) + 623204391074512500*sin(2*q3 + 2*q4 - 2*q5) - 597129945057112500*sin(2*q3 + 2*q4 + 2*q5) + 481743625440000000*sin(3*q3 + 2*q4 - q5) - 13627458640125000*sin(2*q3 + 2*q4 - 3*q5) - 30654966263625000*sin(2*q3 + 2*q4 + 3*q5) + 262162593000000000*sin(3*q3 + 2*q4 - 2*q5) - 262162593000000000*sin(3*q3 + 2*q4 + 2*q5) - 7497244321875000*sin(2*q3 + 2*q4 - 4*q5) + 7497244321875000*sin(2*q3 + 2*q4 + 4*q5) + 1228986628853824500*cos(2*q2 + q3 + q4 - q5) + 434655564841344000*cos(2*q2 + q3 - q4 + q5) - 249133906560000000*cos(2*q2 - q3 + q4 + q5) - 133864358657663700*cos(2*q2 + q3 + q4 - 2*q5) - 76464939583365300*cos(2*q2 + q3 + q4 + 2*q5) + 662959470010363680*cos(2*q2 + 2*q3 + q4 + q5) + 1033973200804500*cos(2*q2 + q3 + q4 - 3*q5) - 10354424545030500*cos(2*q2 + q3 + q4 + 3*q5) + 64908089414784000*cos(2*q2 + q3 + 3*q4 + q5) - 703860871308672000*cos(2*q2 + 3*q3 + q4 + q5) + 2754449762625000*cos(2*q2 + q3 + q4 - 4*q5) + 2754449762625000*cos(2*q2 + q3 + q4 + 4*q5) - 459578782924800000*cos(2*q2 + 4*q3 + q4 + q5) - 307377103638528000*sin(2*q2 + q3 - 2*q4 + q5) + 76749726504528000*sin(2*q2 + q3 + 2*q4 + q5) + 79556426824089600*cos(3*q4 - 2*q5) - 79556426824089600*cos(3*q4 + 2*q5) + 25976537782272000*cos(3*q4 - 3*q5) + 25976537782272000*cos(3*q4 + 3*q5) - 3452951616468750*sin(2*q2 - q5) + 51773906290713750*sin(2*q2 - 2*q5) - 25699460273313750*sin(2*q2 + 2*q5) + 6668652774093750*sin(2*q2 - 3*q5) - 10358854849406250*sin(2*q2 + 3*q5) + 241806438720000000*sin(2*q3 - 2*q5) - 241806438720000000*sin(2*q3 + 2*q5) + 436225685522457600*sin(2*q4 - q5) - 5890691967187500*sin(2*q2 - 4*q5) + 5890691967187500*sin(2*q2 + 4*q5) + 483047341545162240*sin(2*q4 - 2*q5) - 438682456586626560*sin(2*q4 + 2*q5) - 4350407411750400*sin(2*q4 - 3*q5) - 33322199040345600*sin(2*q4 + 3*q5) - 7289334581760000*sin(2*q4 - 4*q5) + 7289334581760000*sin(2*q4 + 4*q5) + 654294339572379000*cos(q3 + q4 - q5) + 263215575638400000*cos(q3 - q4 + q5) + 71554218859200000*cos(2*q2 + q4 + q5) - 205090323780058200*cos(q3 + q4 - 2*q5) - 173037747243259800*cos(q3 + q4 + 2*q5) - 1294599914315400000*cos(2*q3 + q4 + q5) + 52127781457257000*cos(q3 + q4 - 3*q5) + 44535516293367000*cos(q3 + q4 + 3*q5) + 129816178829568000*cos(q3 + 3*q4 + q5) - 747401719680000000*cos(3*q3 + q4 + q5) + 3305339715150000*cos(q3 + q4 - 4*q5) + 3305339715150000*cos(q3 + q4 + 4*q5) + 6892354355040000*sin(2*q2 + q3 + q5) - 204918069092352000*sin(q3 - 2*q4 + q5) + 688511307840972000*sin(q3 + 2*q4 + q5) + 1695144023107956960*cos(q4 + q5) + 434655564841344000*cos(2*q2 + q3 - q4 - q5) - 249133906560000000*cos(2*q2 - q3 + q4 - q5) - 541171909059375000*cos(2*q2 - q3 - q4 + q5) - 99499082360832000*cos(2*q2 + q3 - q4 - 2*q5) - 99499082360832000*cos(2*q2 + q3 - q4 + 2*q5) - 270106914000000000*cos(2*q2 - 2*q3 - q4 + q5) + 659458095958310880*cos(2*q2 + 2*q3 + q4 - q5) + 198288207833210880*cos(2*q2 + 2*q3 - q4 + q5) + 70408345392000000*cos(2*q2 + q3 - q4 - 3*q5) + 70408345392000000*cos(2*q2 + q3 - q4 + 3*q5) + 64908089414784000*cos(2*q2 + q3 + 3*q4 - q5) - 140429041403466816*cos(2*q2 + 2*q3 + q4 - 2*q5) - 57922730157466944*cos(2*q2 + 2*q3 + q4 + 2*q5) - 703860871308672000*cos(2*q2 + 3*q3 + q4 - q5) + 86253779082240000*cos(2*q2 + q3 + 3*q4 - 2*q5) - 86253779082240000*cos(2*q2 + q3 + 3*q4 + 2*q5) - 21687664559631840*cos(2*q2 + 2*q3 + q4 - 3*q5) - 32191786715790240*cos(2*q2 + 2*q3 + q4 + 3*q5) + 98765956556688960*cos(2*q2 + 2*q3 + 3*q4 + q5) - 24874770590208000*cos(2*q2 + 3*q3 + q4 - 2*q5) - 24874770590208000*cos(2*q2 + 3*q3 + q4 + 2*q5) - 459578782924800000*cos(2*q2 + 4*q3 + q4 - q5) + 28163338156800000*cos(2*q2 + q3 + 3*q4 - 3*q5) + 28163338156800000*cos(2*q2 + q3 + 3*q4 + 3*q5) + 2032459871904000*cos(2*q2 + 2*q3 + q4 - 4*q5) + 2032459871904000*cos(2*q2 + 2*q3 + q4 + 4*q5) + 139078540684066500*cos(2*q2 + 3*q3 + 3*q4 + q5) + 100469397659400000*cos(2*q2 + 4*q3 + 3*q4 + q5) + 8026910600940000*sin(q3 + q5) - 307377103638528000*sin(2*q2 + q3 - 2*q4 - q5) + 68897040635808000*sin(2*q2 + q3 + 2*q4 - q5) - 361307719080000000*sin(2*q2 - q3 - 2*q4 + q5) + 267637055938560000*sin(2*q2 + q3 - 2*q4 - 2*q5) - 267637055938560000*sin(2*q2 + q3 - 2*q4 + 2*q5) + 191880299736972000*sin(2*q2 + q3 + 2*q4 - 2*q5) - 155805536776428000*sin(2*q2 + q3 + 2*q4 + 2*q5) - 130574643375000000*sin(2*q2 - 2*q3 - 2*q4 + q5) - 94503391863767040*sin(2*q2 + 2*q3 - 2*q4 + q5) + 79191348804751590*sin(2*q2 + 2*q3 + 2*q4 + q5) + 8375360065380000*sin(2*q2 + q3 + 2*q4 - 3*q5) - 15182697540780000*sin(2*q2 + q3 + 2*q4 + 3*q5) + 576295999026132000*sin(2*q2 + 3*q3 + 2*q4 + q5) - 1975744386000000*sin(2*q2 + q3 + 2*q4 - 4*q5) + 1975744386000000*sin(2*q2 + q3 + 2*q4 + 4*q5) - 5810099146494720*sin(2*q2 + 2*q3 + 4*q4 + q5) + 388795443590400000*sin(2*q2 + 4*q3 + 2*q4 + q5) - 6299214635868000*sin(2*q2 + 3*q3 + 4*q4 + q5) - 6214471984668750*sin(2*q2 + 4*q3 + 4*q4 + q5) + 263215575638400000*cos(q3 - q4 - q5) + 71554218859200000*cos(2*q2 + q4 - q5) - 31194357763800000*cos(2*q2 - q4 + q5) - 74624311770624000*cos(q3 - q4 - 2*q5) - 74624311770624000*cos(q3 - q4 + 2*q5) - 15279452773200000*cos(2*q2 + q4 - 2*q5) - 38658187537200000*cos(2*q2 + q4 + 2*q5) - 1294599914315400000*cos(2*q3 + q4 - q5) - 229789391462400000*cos(2*q3 - q4 + q5) + 42245007235200000*cos(q3 - q4 - 3*q5) + 42245007235200000*cos(q3 - q4 + 3*q5) + 129816178829568000*cos(q3 + 3*q4 - q5) + 22900673565000000*cos(2*q2 + q4 - 3*q5) + 22900673565000000*cos(2*q2 + q4 + 3*q5) + 27887931363600000*cos(2*q3 + q4 - 2*q5) - 135763211984400000*cos(2*q3 + q4 + 2*q5) - 747401719680000000*cos(3*q3 + q4 - q5) + 172507558164480000*cos(q3 + 3*q4 - 2*q5) - 172507558164480000*cos(q3 + 3*q4 + 2*q5) + 68702020695000000*cos(2*q3 + q4 - 3*q5) + 68702020695000000*cos(2*q3 + q4 + 3*q5) + 138200062354200000*cos(2*q3 + 3*q4 + q5) + 56326676313600000*cos(q3 + 3*q4 - 3*q5) + 56326676313600000*cos(q3 + 3*q4 + 3*q5) + 73537762505625000*cos(3*q3 + 3*q4 + q5) + 15333099750698400*sin(q5) - 11430579338640000*sin(2*q2 + q3 - q5) - 188957478197426400*sin(2*q2 + q3 - 2*q5) + 249082083131666400*sin(2*q2 + q3 + 2*q5) + 3782170647763200*sin(2*q2 + 2*q3 + q5) - 204918069092352000*sin(q3 - 2*q4 - q5) + 675423498059772000*sin(q3 + 2*q4 - q5) + 20677063065120000*sin(2*q2 + q3 - 3*q5) - 34291738015920000*sin(2*q2 + q3 + 3*q5) - 444337649817600000*sin(2*q2 - 2*q4 + q5) + 166626618681600000*sin(2*q2 + 2*q4 + q5) + 178424703959040000*sin(q3 - 2*q4 - 2*q5) - 178424703959040000*sin(q3 - 2*q4 + 2*q5) + 655716687068520000*sin(q3 + 2*q4 - 2*q5) - 595592082134280000*sin(q3 + 2*q4 + 2*q5) - 7902977544000000*sin(2*q2 + q3 - 4*q5) + 7902977544000000*sin(2*q2 + q3 + 4*q5) + 965614734321600000*sin(2*q3 + 2*q4 + q5) - 4193966492100000*sin(q3 + 2*q4 - 3*q5) - 43457395835700000*sin(q3 + 2*q4 + 3*q5) + 481743625440000000*sin(3*q3 + 2*q4 + q5) - 9878721930000000*sin(q3 + 2*q4 - 4*q5) + 9878721930000000*sin(q3 + 2*q4 + 4*q5) + 1232782761435769500*cos(2*q2 + q3 + q4 + q5)))/(128*(7263190296986061200*cos(2*q2 + q3) + 235345297533337600*cos(q3 - 2*q4) + 822231539407213600*cos(q3 + 2*q4) - 10296023092740000*cos(q3 - q5) - 2222884258031250*cos(2*q2 + q5) - 70107391443751200*cos(q3 - 2*q5) - 76119851937175200*cos(q3 + 2*q5) + 8026910600940000*cos(q3 - 3*q5) + 10296023092740000*cos(q3 + 3*q5) - 445882949398656000*cos(2*q4 + q5) - 493936096500000*cos(q3 - 4*q5) - 493936096500000*cos(q3 + 4*q5) - 361307719080000000*cos(2*q2 - q3 - 2*q4 - q5) + 131081296500000000*cos(2*q2 - q3 - 2*q4 - 2*q5) + 131081296500000000*cos(2*q2 - q3 - 2*q4 + 2*q5) - 130574643375000000*cos(2*q2 - 2*q3 - 2*q4 - q5) - 94503391863767040*cos(2*q2 + 2*q3 - 2*q4 - q5) + 63858249054053190*cos(2*q2 + 2*q3 + 2*q4 - q5) + 42634860468750000*cos(2*q2 - 2*q3 - 2*q4 - 2*q5) + 42634860468750000*cos(2*q2 - 2*q3 - 2*q4 + 2*q5) + 41142637618790400*cos(2*q2 + 2*q3 - 2*q4 - 2*q5) + 41142637618790400*cos(2*q2 + 2*q3 - 2*q4 + 2*q5) + 117922758939169173*cos(2*q2 + 2*q3 + 2*q4 - 2*q5) + 82703093451201333*cos(2*q2 + 2*q3 + 2*q4 + 2*q5) + 571060875113652000*cos(2*q2 + 3*q3 + 2*q4 - q5) + 9384755223441510*cos(2*q2 + 2*q3 + 2*q4 - 3*q5) + 5948344527256890*cos(2*q2 + 2*q3 + 2*q4 + 3*q5) - 5810099146494720*cos(2*q2 + 2*q3 + 4*q4 - q5) + 179409040132014000*cos(2*q2 + 3*q3 + 2*q4 - 2*q5) + 167384119145166000*cos(2*q2 + 3*q3 + 2*q4 + 2*q5) + 388795443590400000*cos(2*q2 + 4*q3 + 2*q4 - q5) + 374015676035925*cos(2*q2 + 2*q3 + 2*q4 - 4*q5) + 374015676035925*cos(2*q2 + 2*q3 + 2*q4 + 4*q5) - 7501747732617600*cos(2*q2 + 2*q3 + 4*q4 - 2*q5) - 7501747732617600*cos(2*q2 + 2*q3 + 4*q4 + 2*q5) + 2617561956240000*cos(2*q2 + 3*q3 + 2*q4 - 3*q5) + 2617561956240000*cos(2*q2 + 3*q3 + 2*q4 + 3*q5) - 6299214635868000*cos(2*q2 + 3*q3 + 4*q4 - q5) + 96722575488000000*cos(2*q2 + 4*q3 + 2*q4 - 2*q5) + 96722575488000000*cos(2*q2 + 4*q3 + 2*q4 + 2*q5) - 3139383871008000*cos(2*q2 + 2*q3 + 4*q4 - 3*q5) + 3139383871008000*cos(2*q2 + 2*q3 + 4*q4 + 3*q5) - 8133272414190000*cos(2*q2 + 3*q3 + 4*q4 - 2*q5) - 8133272414190000*cos(2*q2 + 3*q3 + 4*q4 + 2*q5) - 6214471984668750*cos(2*q2 + 4*q3 + 4*q4 - q5) - 455583411360000*cos(2*q2 + 2*q3 + 4*q4 - 4*q5) - 455583411360000*cos(2*q2 + 2*q3 + 4*q4 + 4*q5) - 3403668737700000*cos(2*q2 + 3*q3 + 4*q4 - 3*q5) + 3403668737700000*cos(2*q2 + 3*q3 + 4*q4 + 3*q5) - 8111604301453125*cos(2*q2 + 4*q3 + 4*q4 - 2*q5) - 8111604301453125*cos(2*q2 + 4*q3 + 4*q4 + 2*q5) - 493936096500000*cos(2*q2 + 3*q3 + 4*q4 - 4*q5) - 493936096500000*cos(2*q2 + 3*q3 + 4*q4 + 4*q5) - 3075168396093750*cos(2*q2 + 4*q3 + 4*q4 - 3*q5) + 3075168396093750*cos(2*q2 + 4*q3 + 4*q4 + 3*q5) - 401638088671875*cos(2*q2 + 4*q3 + 4*q4 - 4*q5) - 401638088671875*cos(2*q2 + 4*q3 + 4*q4 + 4*q5) + 572253033856000000*sin(q3 - q4) - 158513188718920000*sin(2*q2 + q4) + 2944433354427040000*sin(2*q3 + q4) - 27516460414105600*sin(q3 + 3*q4) - 1693976898423939360*sin(q4 - q5) + 1716759101568000000*sin(3*q3 + q4) + 153879467142538368*sin(q4 - 2*q5) - 54179474609538432*sin(q4 + 2*q5) - 7896057578529120*sin(q4 - 3*q5) + 6728932894511520*sin(q4 + 3*q5) + 59868167177871360*sin(q5 - 3*q4) + 59868167177871360*sin(3*q4 + q5) - 762172451964000*sin(q4 - 4*q5) + 762172451964000*sin(q4 + 4*q5) + 541171909059375000*sin(2*q2 - q3 - q4 - q5) + 20956287886875000*sin(2*q2 - q3 - q4 - 2*q5) - 8282866618125000*sin(2*q2 - q3 - q4 + 2*q5) + 270106914000000000*sin(2*q2 - 2*q3 - q4 - q5) - 198288207833210880*sin(2*q2 + 2*q3 - q4 - q5) - 8276178796875000*sin(2*q2 - q3 - q4 - 3*q5) + 8276178796875000*sin(2*q2 - q3 - q4 + 3*q5) + 22943317814968320*sin(2*q2 + 2*q3 - q4 - 2*q5) - 22943317814968320*sin(2*q2 + 2*q3 - q4 + 2*q5) - 8658845927424000*sin(2*q2 + 2*q3 - q4 - 3*q5) + 8658845927424000*sin(2*q2 + 2*q3 - q4 + 3*q5) - 96431707188653760*sin(2*q2 + 2*q3 + 3*q4 - q5) - 69833941914955680*sin(2*q2 + 2*q3 + 3*q4 - 2*q5) - 68169321819133920*sin(2*q2 + 2*q3 + 3*q4 + 2*q5) - 137813163156751500*sin(2*q2 + 3*q3 + 3*q4 - q5) - 17459528466441600*sin(2*q2 + 2*q3 + 3*q4 - 3*q5) + 15125279098406400*sin(2*q2 + 2*q3 + 3*q4 + 3*q5) - 87935052464349750*sin(2*q2 + 3*q3 + 3*q4 - 2*q5) - 87032675499140250*sin(2*q2 + 3*q3 + 3*q4 + 2*q5) - 100469397659400000*sin(2*q2 + 4*q3 + 3*q4 - q5) - 254057483988000*sin(2*q2 + 2*q3 + 3*q4 - 4*q5) + 254057483988000*sin(2*q2 + 2*q3 + 3*q4 + 4*q5) - 18296646946132500*sin(2*q2 + 3*q3 + 3*q4 - 3*q5) + 17031269418817500*sin(2*q2 + 3*q3 + 3*q4 + 3*q5) - 58446836910000000*sin(2*q2 + 4*q3 + 3*q4 - 2*q5) - 58446836910000000*sin(2*q2 + 4*q3 + 3*q4 + 2*q5) - 137722488131250*sin(2*q2 + 3*q3 + 3*q4 - 4*q5) + 137722488131250*sin(2*q2 + 3*q3 + 3*q4 + 4*q5) - 10178077140000000*sin(2*q2 + 4*q3 + 3*q4 - 3*q5) + 10178077140000000*sin(2*q2 + 4*q3 + 3*q4 + 3*q5) + 656825094627009000*sin(q3 + q4 + q5) + 2484582864105156250*cos(2*q2) - 4926469791532800000*cos(2*q3) - 2367527063552000000*cos(3*q3) + 588766372249655040*cos(2*q4) - 427286086914756762*cos(2*q5) + 15333099750698400*cos(3*q5) + 1659198174791850*cos(4*q5) + 362523922404000000*cos(2*q2 - q3 - 2*q4) + 52432518600000000*cos(2*q2 - q3 - 2*q5) + 52432518600000000*cos(2*q2 - q3 + 2*q5) + 121539759200000000*cos(2*q2 - 2*q3 - 2*q4) + 108535713685962752*cos(2*q2 + 2*q3 - 2*q4) + 219268169384091360*cos(2*q2 + 2*q3 + 2*q4) - 5875093228435200*cos(2*q2 + 2*q3 - q5) - 65734904324251008*cos(2*q2 + 2*q3 - 2*q5) - 87917346803518848*cos(2*q2 + 2*q3 + 2*q5) + 506145222779579600*cos(2*q2 + 3*q3 + 2*q4) - 444337649817600000*cos(2*q2 - 2*q4 - q5) + 166626618681600000*cos(2*q2 + 2*q4 - q5) + 4766264781884032*cos(2*q2 + 2*q3 + 4*q4) + 3782170647763200*cos(2*q2 + 2*q3 - 3*q5) + 5875093228435200*cos(2*q2 + 2*q3 + 3*q5) + 181354829040000000*cos(2*q2 - 2*q4 - 2*q5) + 181354829040000000*cos(2*q2 - 2*q4 + 2*q5) + 60451609680000000*cos(2*q2 + 2*q4 - 2*q5) + 60451609680000000*cos(2*q2 + 2*q4 + 2*q5) + 301441812891520000*cos(2*q2 + 4*q3 + 2*q4) + 959938898447100000*cos(2*q3 + 2*q4 - q5) - 911166822720000*cos(2*q2 + 2*q3 - 4*q5) - 911166822720000*cos(2*q2 + 2*q3 + 4*q5) + 5167506459950800*cos(2*q2 + 3*q3 + 4*q4) + 311602195537256250*cos(2*q3 + 2*q4 - 2*q5) + 298564972528556250*cos(2*q3 + 2*q4 + 2*q5) + 481743625440000000*cos(3*q3 + 2*q4 - q5) + 6747481134426250*cos(2*q2 + 4*q3 + 4*q4) - 4542486213375000*cos(2*q3 + 2*q4 - 3*q5) + 10218322087875000*cos(2*q3 + 2*q4 + 3*q5) + 131081296500000000*cos(3*q3 + 2*q4 - 2*q5) + 131081296500000000*cos(3*q3 + 2*q4 + 2*q5) - 1874311080468750*cos(2*q3 + 2*q4 - 4*q5) - 1874311080468750*cos(2*q3 + 2*q4 + 4*q5) - 12689944096858112*sin(3*q4) - 1249392186595000000*sin(2*q2 - q3 - q4) - 620427396400000000*sin(2*q2 - 2*q3 - q4) + 435572897953292288*sin(2*q2 + 2*q3 - q4) + 31194357763800000*sin(2*q2 - q4 - q5) - 31837535762018112*sin(2*q2 + 2*q3 + 3*q4) + 46297913923800000*sin(2*q2 - q4 - 2*q5) - 34608546541800000*sin(2*q2 - q4 + 2*q5) + 229789391462400000*sin(2*q3 - q4 - q5) - 22900673565000000*sin(2*q2 - q4 - 3*q5) + 22900673565000000*sin(2*q2 - q4 + 3*q5) - 17256978940052800*sin(2*q2 + 3*q3 + 3*q4) + 1004061914520000*sin(2*q2 + 4*q3 + 3*q4) - 138200062354200000*sin(2*q3 + 3*q4 - q5) - 87670255365000000*sin(2*q3 + 3*q4 - 2*q5) - 87670255365000000*sin(2*q3 + 3*q4 + 2*q5) - 73537762505625000*sin(3*q3 + 3*q4 - q5) - 17811634995000000*sin(2*q3 + 3*q4 - 3*q5) + 17811634995000000*sin(2*q3 + 3*q4 + 3*q5) - 44356974440625000*sin(3*q3 + 3*q4 - 2*q5) - 44356974440625000*sin(3*q3 + 3*q4 + 2*q5) - 8276178796875000*sin(3*q3 + 3*q4 - 3*q5) + 8276178796875000*sin(3*q3 + 3*q4 + 3*q5) + 307377103638528000*cos(2*q2 + q3 - 2*q4 + q5) - 76749726504528000*cos(2*q2 + q3 + 2*q4 + q5) - 1228986628853824500*sin(2*q2 + q3 + q4 - q5) + 434655564841344000*sin(2*q2 + q3 - q4 + q5) - 249133906560000000*sin(2*q2 - q3 + q4 + q5) + 66932179328831850*sin(2*q2 + q3 + q4 - 2*q5) - 38232469791682650*sin(2*q2 + q3 + q4 + 2*q5) + 662959470010363680*sin(2*q2 + 2*q3 + q4 + q5) - 344657733601500*sin(2*q2 + q3 + q4 - 3*q5) - 3451474848343500*sin(2*q2 + q3 + q4 + 3*q5) + 64908089414784000*sin(2*q2 + q3 + 3*q4 + q5) - 703860871308672000*sin(2*q2 + 3*q3 + q4 + q5) - 688612440656250*sin(2*q2 + q3 + q4 - 4*q5) + 688612440656250*sin(2*q2 + q3 + q4 + 4*q5) - 459578782924800000*sin(2*q2 + 4*q3 + q4 + q5) - 2505845877220000000*cos(2*q2 - q3) - 1283417094400000000*cos(2*q2 - 2*q3) + 2481886935200625792*cos(2*q2 + 2*q3) - 2160642062805811200*cos(2*q2 + 3*q3) + 486134414554880000*cos(2*q2 - 2*q4) + 167187503038080000*cos(2*q2 + 2*q4) - 3452951616468750*cos(2*q2 - q5) - 1091847775191040000*cos(2*q2 + 4*q3) + 25886953145356875*cos(2*q2 - 2*q5) + 12849730136656875*cos(2*q2 + 2*q5) + 883398735766092500*cos(2*q3 + 2*q4) + 2222884258031250*cos(2*q2 - 3*q5) + 3452951616468750*cos(2*q2 + 3*q5) + 120903219360000000*cos(2*q3 - 2*q5) + 120903219360000000*cos(2*q3 + 2*q5) + 395977698872000000*cos(3*q3 + 2*q4) + 436225685522457600*cos(2*q4 - q5) - 1472672991796875*cos(2*q2 - 4*q5) - 1472672991796875*cos(2*q2 + 4*q5) + 241523670772581120*cos(2*q4 - 2*q5) + 219341228293313280*cos(2*q4 + 2*q5) - 1450135803916800*cos(2*q4 - 3*q5) + 11107399680115200*cos(2*q4 + 3*q5) - 1822333645440000*cos(2*q4 - 4*q5) - 1822333645440000*cos(2*q4 + 4*q5) - 112565280336880000*sin(2*q2 - q4) - 527819268874240000*sin(2*q3 - q4) - 18143529750640000*sin(2*q3 + 3*q4) - 3498748733000000*sin(3*q3 + 3*q4) - 39778213412044800*sin(3*q4 - 2*q5) - 39778213412044800*sin(3*q4 + 2*q5) - 8658845927424000*sin(3*q4 - 3*q5) + 8658845927424000*sin(3*q4 + 3*q5) - 6892354355040000*cos(2*q2 + q3 + q5) + 204918069092352000*cos(q3 - 2*q4 + q5) - 688511307840972000*cos(q3 + 2*q4 + q5) - 2802173268057527600*sin(2*q2 + q3 + q4) - 654294339572379000*sin(q3 + q4 - q5) + 263215575638400000*sin(q3 - q4 + q5) + 71554218859200000*sin(2*q2 + q4 + q5) + 102545161890029100*sin(q3 + q4 - 2*q5) - 86518873621629900*sin(q3 + q4 + 2*q5) - 1294599914315400000*sin(2*q3 + q4 + q5) - 17375927152419000*sin(q3 + q4 - 3*q5) + 14845172097789000*sin(q3 + q4 + 3*q5) + 129816178829568000*sin(q3 + 3*q4 + q5) - 747401719680000000*sin(3*q3 + q4 + q5) - 826334928787500*sin(q3 + q4 - 4*q5) + 826334928787500*sin(q3 + q4 + 4*q5) - 8026910600940000*cos(q3 + q5) - 307377103638528000*cos(2*q2 + q3 - 2*q4 - q5) + 68897040635808000*cos(2*q2 + q3 + 2*q4 - q5) + 361307719080000000*cos(2*q2 - q3 - 2*q4 + q5) + 133818527969280000*cos(2*q2 + q3 - 2*q4 - 2*q5) + 133818527969280000*cos(2*q2 + q3 - 2*q4 + 2*q5) + 95940149868486000*cos(2*q2 + q3 + 2*q4 - 2*q5) + 77902768388214000*cos(2*q2 + q3 + 2*q4 + 2*q5) + 130574643375000000*cos(2*q2 - 2*q3 - 2*q4 + q5) + 94503391863767040*cos(2*q2 + 2*q3 - 2*q4 + q5) - 79191348804751590*cos(2*q2 + 2*q3 + 2*q4 + q5) + 2791786688460000*cos(2*q2 + q3 + 2*q4 - 3*q5) + 5060899180260000*cos(2*q2 + q3 + 2*q4 + 3*q5) - 576295999026132000*cos(2*q2 + 3*q3 + 2*q4 + q5) - 493936096500000*cos(2*q2 + q3 + 2*q4 - 4*q5) - 493936096500000*cos(2*q2 + q3 + 2*q4 + 4*q5) + 5810099146494720*cos(2*q2 + 2*q3 + 4*q4 + q5) - 388795443590400000*cos(2*q2 + 4*q3 + 2*q4 + q5) + 6299214635868000*cos(2*q2 + 3*q3 + 4*q4 + q5) + 6214471984668750*cos(2*q2 + 4*q3 + 4*q4 + q5) - 1452769072173234800*sin(q3 + q4) + 1695144023107956960*sin(q4 + q5) - 434655564841344000*sin(2*q2 + q3 - q4 - q5) + 249133906560000000*sin(2*q2 - q3 + q4 - q5) - 541171909059375000*sin(2*q2 - q3 - q4 + q5) + 49749541180416000*sin(2*q2 + q3 - q4 - 2*q5) - 49749541180416000*sin(2*q2 + q3 - q4 + 2*q5) - 270106914000000000*sin(2*q2 - 2*q3 - q4 + q5) - 659458095958310880*sin(2*q2 + 2*q3 + q4 - q5) + 198288207833210880*sin(2*q2 + 2*q3 - q4 + q5) - 23469448464000000*sin(2*q2 + q3 - q4 - 3*q5) + 23469448464000000*sin(2*q2 + q3 - q4 + 3*q5) - 64908089414784000*sin(2*q2 + q3 + 3*q4 - q5) + 70214520701733408*sin(2*q2 + 2*q3 + q4 - 2*q5) - 28961365078733472*sin(2*q2 + 2*q3 + q4 + 2*q5) + 703860871308672000*sin(2*q2 + 3*q3 + q4 - q5) - 43126889541120000*sin(2*q2 + q3 + 3*q4 - 2*q5) - 43126889541120000*sin(2*q2 + q3 + 3*q4 + 2*q5) + 7229221519877280*sin(2*q2 + 2*q3 + q4 - 3*q5) - 10730595571930080*sin(2*q2 + 2*q3 + q4 + 3*q5) + 98765956556688960*sin(2*q2 + 2*q3 + 3*q4 + q5) + 12437385295104000*sin(2*q2 + 3*q3 + q4 - 2*q5) - 12437385295104000*sin(2*q2 + 3*q3 + q4 + 2*q5) + 459578782924800000*sin(2*q2 + 4*q3 + q4 - q5) - 9387779385600000*sin(2*q2 + q3 + 3*q4 - 3*q5) + 9387779385600000*sin(2*q2 + q3 + 3*q4 + 3*q5) - 508114967976000*sin(2*q2 + 2*q3 + q4 - 4*q5) + 508114967976000*sin(2*q2 + 2*q3 + q4 + 4*q5) + 139078540684066500*sin(2*q2 + 3*q3 + 3*q4 + q5) + 100469397659400000*sin(2*q2 + 4*q3 + 3*q4 + q5) + 5029599035533917600*cos(q3) - 15333099750698400*cos(q5) + 353017946300006400*cos(2*q2 + q3 - 2*q4) + 195374268399248400*cos(2*q2 + q3 + 2*q4) - 11430579338640000*cos(2*q2 + q3 - q5) - 94478739098713200*cos(2*q2 + q3 - 2*q5) - 124541041565833200*cos(2*q2 + q3 + 2*q5) - 3782170647763200*cos(2*q2 + 2*q3 + q5) - 204918069092352000*cos(q3 - 2*q4 - q5) + 675423498059772000*cos(q3 + 2*q4 - q5) + 6892354355040000*cos(2*q2 + q3 - 3*q5) + 11430579338640000*cos(2*q2 + q3 + 3*q5) + 444337649817600000*cos(2*q2 - 2*q4 + q5) - 166626618681600000*cos(2*q2 + 2*q4 + q5) + 89212351979520000*cos(q3 - 2*q4 - 2*q5) + 89212351979520000*cos(q3 - 2*q4 + 2*q5) + 327858343534260000*cos(q3 + 2*q4 - 2*q5) + 297796041067140000*cos(q3 + 2*q4 + 2*q5) - 1975744386000000*cos(2*q2 + q3 - 4*q5) - 1975744386000000*cos(2*q2 + q3 + 4*q5) - 965614734321600000*cos(2*q3 + 2*q4 + q5) - 1397988830700000*cos(q3 + 2*q4 - 3*q5) + 14485798611900000*cos(q3 + 2*q4 + 3*q5) - 481743625440000000*cos(3*q3 + 2*q4 + q5) - 2469680482500000*cos(q3 + 2*q4 - 4*q5) - 2469680482500000*cos(q3 + 2*q4 + 4*q5) - 3775857455561867648*sin(q4) + 944482049133414400*sin(2*q2 + q3 - q4) + 572253033856000000*sin(2*q2 - q3 + q4) - 1498149960073735360*sin(2*q2 + 2*q3 + q4) - 263215575638400000*sin(q3 - q4 - q5) - 13758230207052800*sin(2*q2 + q3 + 3*q4) - 71554218859200000*sin(2*q2 + q4 - q5) - 31194357763800000*sin(2*q2 - q4 + q5) + 1616747092278707200*sin(2*q2 + 3*q3 + q4) + 37312155885312000*sin(q3 - q4 - 2*q5) - 37312155885312000*sin(q3 - q4 + 2*q5) + 7639726386600000*sin(2*q2 + q4 - 2*q5) - 19329093768600000*sin(2*q2 + q4 + 2*q5) + 1055638537748480000*sin(2*q2 + 4*q3 + q4) + 1294599914315400000*sin(2*q3 + q4 - q5) - 229789391462400000*sin(2*q3 - q4 + q5) - 14081669078400000*sin(q3 - q4 - 3*q5) + 14081669078400000*sin(q3 - q4 + 3*q5) - 129816178829568000*sin(q3 + 3*q4 - q5) - 7633557855000000*sin(2*q2 + q4 - 3*q5) + 7633557855000000*sin(2*q2 + q4 + 3*q5) - 13943965681800000*sin(2*q3 + q4 - 2*q5) - 67881605992200000*sin(2*q3 + q4 + 2*q5) + 747401719680000000*sin(3*q3 + q4 - q5) - 86253779082240000*sin(q3 + 3*q4 - 2*q5) - 86253779082240000*sin(q3 + 3*q4 + 2*q5) - 22900673565000000*sin(2*q3 + q4 - 3*q5) + 22900673565000000*sin(2*q3 + q4 + 3*q5) + 138200062354200000*sin(2*q3 + 3*q4 + q5) - 18775558771200000*sin(q3 + 3*q4 - 3*q5) + 18775558771200000*sin(q3 + 3*q4 + 3*q5) + 73537762505625000*sin(3*q3 + 3*q4 + q5) + 1232782761435769500*sin(2*q2 + q3 + q4 + q5) + 7646094127248401852)^(1/2));
%     0];

%% %% Reduntant Controller
%% manipulability measure #2: W=1/2*(sin(qi)^2)
kp=10;
dq0=[-cos(q5)*sin(q5), cos(q2)*sin(q2), cos(q3)*sin(q3), cos(q4)*sin(q4), -cos(q5)*sin(q5), 0].' ;
%cos(q6)*sin(q6) ,no need to add since it has no effect.


%% Inverse Kinematic Controller
K = kp*eye(3);
P=eye(6)-pinv(Jp)*Jp;
dq=pinv(Jp)*(xd_des+K*(x_des-x))+100*P*dq0;
